simulink model "IEEE34bus_LeonardoEdit_Phasor_PI_ZIPload"  (R2024a)
settings: Solver=ode4  StartTime=0.0  StopTime=100  FixedStep=Ts  MaxStep=1e-4  RelTol=1e-4
InitFcn:
  | a=1; % Loading Factor
  | Ts=0.1;% For Delay Blocks in Voltage Regulator Controls
  | % phase to sequence conversion of RXB matrices
  | c=1*exp(sqrt(-1)*(120*pi/180));
  | T=[1 1 1;1 c*c c;1 c c*c];
  | Tinv=1/3*[1 1 1;1 c c*c;1 c*c c];
  | 
  | % Simulation data for the IEEE 34 Node Test Feeder model
  | mi2km = 1.60934;%  miles to km conversion
  | ft2km = 0.0003048; % feet to km conversion
  | ms2F = 1*1e-6/(2*pi*60);% microsiemens to Farads conversion
  | 
  | %% Configuration 300 - series reactance - ohm/mile
  | R_300 = [1.3368 0.2101 0.2130;0.2101 1.3238 0.2066;0.2130 0.2066 1.3294];
  | X_300 = [1.3343 0.5779 0.5015;0.5779 1.3569 0.4591;0.5015 0.4591 1.3471];
  | % charging susceptance - microsiemens/mile
  | B_300 = [5.3350 -1.5313 -0.9943;-1.5313 5.0979 -0.6212;-0.9943 -0.6212 4.8880];
  | 
  | R_300 = R_300/mi2km;
  | Rseq=Tinv*R_300*T;
  | R1_300=Rseq(2,2);R0_300=Rseq(1,1);
  | 
  | L_300 = (X_300/(2*pi*60))/mi2km;
  | Lseq=Tinv*L_300*T;
  | L1_300=Lseq(2,2);L0_300=Lseq(1,1);
  | 
  | C_300 =(B_300*ms2F)/mi2km;
  | Cseq=Tinv*C_300*T;
  | C1_300=Cseq(2,2);C0_300=Cseq(1,1);
  | 
  | %% Configuration 301 - series reactance - ohm/mile
  | R_301 = [1.9300 0.2327 0.2359;0.2327 1.9157 0.2288;0.2359 0.2288 1.9219];
  | X_301 = [1.4115 0.6442 0.5691;0.6442 1.4281 0.5238;0.5691 0.5238 1.4209];
  | % charging susceptance - microsiemens/mile
  | B_301 = [5.1207 -1.4364 -0.9402;-1.4364 4.9055 -0.5951;-0.9402 -0.5951 4.7154];
  | 
  | R_301 = R_301/mi2km;
  | Rseq=Tinv*R_301*T;
  | R1_301=Rseq(2,2);R0_301=Rseq(1,1);
  | 
  | L_301 = (X_301/(2*pi*60))/mi2km;
  | Lseq=Tinv*L_301*T;
  | L1_301=Lseq(2,2);L0_301=Lseq(1,1);
  | 
  | C_301 =(B_301*ms2F)/mi2km;
  | Cseq=Tinv*C_301*T;
  | C1_301=Cseq(2,2);C0_301=Cseq(1,1);
  | 
  | %% Configuration 302 - series reactance - ohm/mile
  | R_302 = [2.7995 0 0;0 0 0;0 0 0];
  | X_302 = [1.4855 0 0;0 0 0;0 0 0];
  | % charging susceptance - microsiemens/mile
  | B_302 = [4.2251 0 0;0 0 0;0 0 0];
  | 
  | R_302 = R_302/mi2km;
  | Rseq=Tinv*R_302*T;
  | R1_302=Rseq(2,2);R0_302=Rseq(1,1);
  | 
  | L_302 = (X_302/(2*pi*60))/mi2km;
  | Lseq=Tinv*L_302*T;
  | L1_302=Lseq(2,2);L0_302=Lseq(1,1);
  | 
  | C_302 =(B_302*ms2F)/mi2km;
  | Cseq=Tinv*C_302*T;
  | C1_302=Cseq(2,2);C0_302=Cseq(1,1);
  | 
  | %% Configuration 303 - series reactance - ohm/mile
  | R_303 = [0 0 0;0 2.7995 0;0 0 0];
  | X_303 = [0 0 0;0 1.4855 0;0 0 0];
  | % charging susceptance - microsiemens/mile
  | B_303 = [0 0 0;0 4.2251 0;0 0 0];
  | 
  | R_303 = R_303/mi2km;
  | Rseq=Tinv*R_303*T;
  | R1_303=Rseq(2,2);R0_303=Rseq(1,1);
  | 
  | L_303 = (X_303/(2*pi*60))/mi2km;
  | Lseq=Tinv*L_303*T;
  | L1_303=Lseq(2,2);L0_303=Lseq(1,1);
  | 
  | C_303 =(B_303*ms2F)/mi2km;
  | Cseq=Tinv*C_303*T;
  | C1_303=Cseq(2,2);C0_303=Cseq(1,1);
  | 
  | %% Configuration 303 - series reactance - ohm/mile
  | R_304 = [0 0 0;0 1.9217 0;0 0 0];
  | X_304 = [0 0 0;0 1.4212 0;0 0 0];
  | % charging susceptance - microsiemens/mile
  | B_304 = [0 0 0;0 4.3637 0;0 0 0];
  | 
  | R_304 = R_304/mi2km;
  | Rseq=Tinv*R_304*T;
  | R1_304=Rseq(2,2);R0_304=Rseq(1,1);
  | 
  | L_304 = (X_304/(2*pi*60))/mi2km;
  | Lseq=Tinv*L_304*T;
  | L1_304=Lseq(2,2);L0_304=Lseq(1,1);
  | 
  | C_304 =(B_304*ms2F)/mi2km;
  | Cseq=Tinv*C_304*T;
  | C1_304=Cseq(2,2);C0_304=Cseq(1,1);
undefined symbols (not defined in the file or in its folder): find_system, j
libraries: spsSeriesRLCBranchLib x157, spsGroundLib x103, spsVoltageMeasurementLib x100, spsControlledCurrentSourceLib x94, spsThreePhaseVIMeasurementLib x37, spsThreePhasePISectionLineLib x20, spsCurrentMeasurementLib x12, spsOnDelayLib x12, spsPiSectionLineLib x8, spsControlledVoltageSourceLib x6, spsDiscreteVariableTimeDelayLib x6, spsMutualInductanceLib x4
(part 1 of 8)
settings Model: ARTEMISmethode_block_infos=$$__separator__$$pi34variableloadwith3PV/ARTEMIS Guide$$__separator__$$  Creator=Arun  LastModifiedBy=leonardofdsantos
settings SolverCC: ShapePreserveControl=EnableAll  AlgebraicLoopSolver=TrustRegion  SolverResetMethod=Robust
settings DataIOCC: ReturnWorkspaceOutputs=off
settings DebuggingCC: ArithmeticOperatorsInVariantConditions=warning
settings ModelReferenceCC: EnableRefExpFcnMdlSchedulingChecks=on
settings SFSimCC: SimUseLocalCustomCode=off  CustomCodeUndefinedFunction=UseInterfaceOnly
settings RTWCC: RTWUseLocalCustomCode=off  GPUComputeCapability=3.5
settings CodeAppCC: StateflowObjectComments=on
settings SimscapeCC: SimscapeNormalizeSystem=off

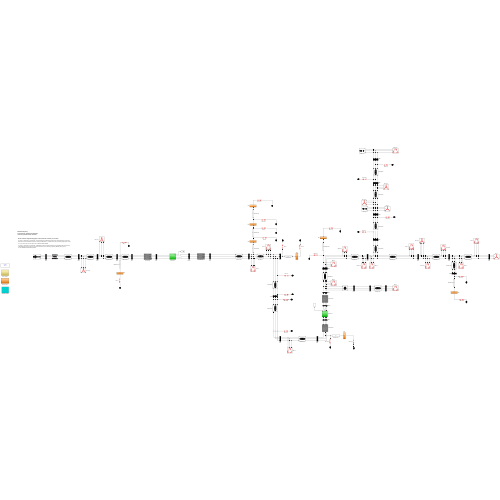
[thumbnail: Simulink's stored preview of the top-level diagram]
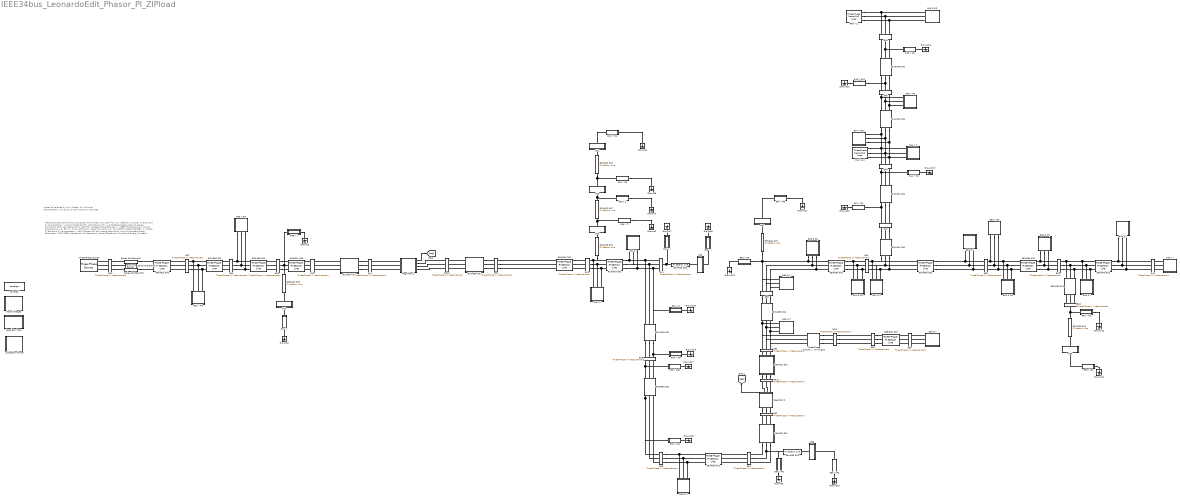
== system IEEE34bus_LeonardoEdit_Phasor_PI_ZIPload ==
  note: Model Developed by
      | Arun Suresh, Dr. Sukumar Kamalasadan,
      | University of North Carolina, Charlotte
  note: Please consider citing following papers if the model was useful for your research
      |
      | A. Suresh, R. Bisht and S. Kamalasadan, "A Coordinated Control Architecture With Inverter-Based Resources and Legacy
      | Controllers of Power Distribution System for Voltage Profile Balance," in IEEE Transactions on Industry Applications, vol. 58,
      | no. 5, pp. 6701-6712, Sept.-Oct. 2022, doi: 10.1109/TIA.2022.3183030.
      |
      | A. Suresh, R. Bisht and S. Kamalasadan, "ADMM Based LQR for Voltage Regulation Using Distributed Energy Resources,"
      | 2020 IEEE International Conference on Power Electronics, Drives and Energy Systems (PEDES), 2020, pp. 1-6,
      | doi: 10.1109/PEDES49360.2020.9379625.
  800 : spsThreePhaseVIMeasurementLib/Three-Phase V-I Measurement  VoltageMeasurement=phase-to-ground  SetLabelV=on  LabelV=V800  Vpu=off  VpuLL=off  CurrentMeasurement=yes  SetLabelI=on  LabelI=I800  Ipu=off  Pbase=100e6  Vbase=24900  OutputType=Complex  PhasorSimulation=on  PSBequivalent=0
  800-802 300 : spsThreePhasePISectionLineLib/Three-Phase PI Section Line  LConnTagsString=a|b|c  RConnTagsString=A|B|C  Length=2580*ft2km  Frequency=60  Resistances=[R1_300 R0_300]  Inductances=[L1_300 L0_300]  Capacitances=[C1_300 C0_300]
  802 : spsThreePhaseVIMeasurementLib/Three-Phase V-I Measurement  VoltageMeasurement=phase-to-ground  SetLabelV=on  LabelV=V802  Vpu=off  VpuLL=off  CurrentMeasurement=yes  SetLabelI=on  LabelI=I802  Ipu=off  Pbase=100e6  Vbase=24900  OutputType=Complex  PhasorSimulation=on  PSBequivalent=0
  802 Y PQ : Subsystem  mask(Three Phase Star ZIP Load (Phasor)){Vnom=24900, fnom=60, Pnom=[1e-6  30 25]*1e3/2 *a, Qnom=[0 15 14]*1e3/2 *a, LoadType=Constant P, Vlim=0.7}
      mask prompts: Vnom "Nominal Ph-Ph voltage (Vrms)"; fnom "Nominal Frequency fn (Hz)"; Pnom "Nominal Per Phase Active Power [Pa Pb Pc] (W)"; Qnom "Nominal Per Phase Reactive Power [Qa Qb Qc] (VAR)"; LoadType "Load Type"; Vlim "Minimum voltage (pu)"
      mask help:
      | Notes:
      | Three Phase Star Connected ZIP load model which gets converted to constant Z type if the voltage becomes lower than the Minimum Voltage.
      mask TypeOptions LoadType: Constant Z | Constant I | Constant P
      mask DialogControl ParameterTabVar0 Prompt: Parameters
      mask DialogControl ParameterTabVar01 Prompt: Type
      mask Display:
      | color('red');
      | %load figure 0deg
      | A=[-210,-180,-170,-160,-147,-140,-130,-120,-110,-80,-50,-49,-45,-39,-33,-26,-21,-18,-17,-19,-22,-22,-26,-27,-25,-22,-16,-9,-3,2,6,6,4,1,1,-3,-4,-2,2,7,14,20,26,29,30,28,24,24,21,20,21,25,31,37,44,49,50,50,80];
      | B=[-41.5,-41.5,-63,-20,-63,-20,-63,-20,-41.5,-41.5,-41.5,-34,-26,-21,-20,-22,-28,-37,-47,-57,-63,-63,-54,-44,-34,-26,-21,-20,-22,-28,-37,-47,-57,-63,-63,-54,-44,-34,-26,-21,-20,-22,-28,-37,-47,-57,-63,-63,-54,-44,-34,-26,-21,-20,-22,-28,-37,-41.50,-41.5];
      | % plot(A,B);
      | 
      | %load figure 0deg inverted
      | A1=[-80,-50,-49,-45,-39,-33,-26,-21,-18,-17,-19,-22,-22,-26,-27,-25,-22,-16,-9,-3,2,6,6,4,1,1,-3,-4,-2,2,7,14,20,26,29,30,28,24,24,21,20,21,25,31,37,44,49,50,50,80,110,120,130,143,150,160,170,180,210];
      | B1=[-41.5,-41.5,-34,-26,-21,-20,-22,-28,-37,-47,-57,-63,-63,-54,-44,-34,-26,-21,-20,-22,-28,-37,-47,-57,-63,-63,-54,-44,-34,-26,-21,-20,-22,-28,-37,-47,-57,-63,-63,-54,-44,-34,-26,-21,-20,-22,-28,-37,-41.5,-41.5,-41.5,-63,-20,-63,-20,-63,-20,-41.5,-41.5];
      | 
      | 
      | %load figure 90deg
      | C=[-41.5,-41.5,-20,-63,-20,-63,-20,-63,-41.5,-41.5,-41.5,-37,-28,-22,-20,-21,-26,-34,-44,-54,-63,-63,-57,-47,-37,-28,-22,-20,-21,-26,-34,-44,-54,-63,-63,-57,-47,-37,-28,-22,-20,-21,-26,-34,-44,-54,-63,-63,-57,-47,-37,-28,-22,-20,-21,-26,-34,-41.5,-41.5];
      | D=[190,160,150,140,130,123,110,100,90,80,50,50,49,44,37,31,25,21,20,21,24,24,28,30,29,26,20,14,7,2,-2,-4,-3,1,1,4,6,6,2,-3,-9,-16,-22,-25,-27,-26,-22,-22,-19,-17,-18,-21,-26,-33,-39,-45,-49,-50,-70];
      | plot(C,D);
      | 
      | 
      | %load figure -120deg
      | c=1*exp(sqrt(-1)*(-60*pi/180));
      | l=A1+j*B1;
      | m=l*c;
      | E=real(m);F=imag(m);
      | E=E+34.4400;F=F-118.53;
      | plot(E,F);
      | 
      | %load figure +120deg
      | c=1*exp(sqrt(-1)*(60*pi/180));
      | l=A+j*B;
      | m=l*c;
      | G=real(m);
      | H=imag(m);
      | G=G-117.44;H=H-118.5300;
      | plot(G,H);
      | 
      | color('black');
      | port_label('LConn', 1, 'A')
      | port_label('LConn', 2, 'B')
      | port_label('LConn', 3, 'C')
  802-806 300 : spsThreePhasePISectionLineLib/Three-Phase PI Section Line  LConnTagsString=a|b|c  RConnTagsString=A|B|C  Length=1730*ft2km  Frequency=60  Resistances=[R1_300 R0_300]  Inductances=[L1_300 L0_300]  Capacitances=[C1_300 C0_300]
  806 : spsThreePhaseVIMeasurementLib/Three-Phase V-I Measurement  VoltageMeasurement=phase-to-ground  SetLabelV=on  LabelV=V806  Vpu=off  VpuLL=off  CurrentMeasurement=yes  SetLabelI=on  LabelI=I806  Ipu=off  Pbase=100e6  Vbase=24900  OutputType=Complex  PhasorSimulation=on  PSBequivalent=0
  806 Y PQ : Subsystem  mask(Three Phase Star ZIP Load (Phasor)){Vnom=24900, fnom=60, Pnom=[1e-6  30 25]*1e3/2 *a, Qnom=[0 15 14]*1e3/2 *a, LoadType=Constant P, Vlim=0.7}
      mask prompts: Vnom "Nominal Ph-Ph voltage (Vrms)"; fnom "Nominal Frequency fn (Hz)"; Pnom "Nominal Per Phase Active Power [Pa Pb Pc] (W)"; Qnom "Nominal Per Phase Reactive Power [Qa Qb Qc] (VAR)"; LoadType "Load Type"; Vlim "Minimum voltage (pu)"
      mask help:
      | Notes:
      | Three Phase Star Connected ZIP load model which gets converted to constant Z type if the voltage becomes lower than the Minimum Voltage.
      mask TypeOptions LoadType: Constant Z | Constant I | Constant P
      mask DialogControl ParameterTabVar0 Prompt: Parameters
      mask DialogControl ParameterTabVar01 Prompt: Type
      mask Display:
      | color('red');
      | %load figure 0deg
      | A=[-210,-180,-170,-160,-147,-140,-130,-120,-110,-80,-50,-49,-45,-39,-33,-26,-21,-18,-17,-19,-22,-22,-26,-27,-25,-22,-16,-9,-3,2,6,6,4,1,1,-3,-4,-2,2,7,14,20,26,29,30,28,24,24,21,20,21,25,31,37,44,49,50,50,80];
      | B=[-41.5,-41.5,-63,-20,-63,-20,-63,-20,-41.5,-41.5,-41.5,-34,-26,-21,-20,-22,-28,-37,-47,-57,-63,-63,-54,-44,-34,-26,-21,-20,-22,-28,-37,-47,-57,-63,-63,-54,-44,-34,-26,-21,-20,-22,-28,-37,-47,-57,-63,-63,-54,-44,-34,-26,-21,-20,-22,-28,-37,-41.50,-41.5];
      | % plot(A,B);
      | 
      | %load figure 0deg inverted
      | A1=[-80,-50,-49,-45,-39,-33,-26,-21,-18,-17,-19,-22,-22,-26,-27,-25,-22,-16,-9,-3,2,6,6,4,1,1,-3,-4,-2,2,7,14,20,26,29,30,28,24,24,21,20,21,25,31,37,44,49,50,50,80,110,120,130,143,150,160,170,180,210];
      | B1=[-41.5,-41.5,-34,-26,-21,-20,-22,-28,-37,-47,-57,-63,-63,-54,-44,-34,-26,-21,-20,-22,-28,-37,-47,-57,-63,-63,-54,-44,-34,-26,-21,-20,-22,-28,-37,-47,-57,-63,-63,-54,-44,-34,-26,-21,-20,-22,-28,-37,-41.5,-41.5,-41.5,-63,-20,-63,-20,-63,-20,-41.5,-41.5];
      | 
      | 
      | %load figure 90deg
      | C=[-41.5,-41.5,-20,-63,-20,-63,-20,-63,-41.5,-41.5,-41.5,-37,-28,-22,-20,-21,-26,-34,-44,-54,-63,-63,-57,-47,-37,-28,-22,-20,-21,-26,-34,-44,-54,-63,-63,-57,-47,-37,-28,-22,-20,-21,-26,-34,-44,-54,-63,-63,-57,-47,-37,-28,-22,-20,-21,-26,-34,-41.5,-41.5];
      | D=[190,160,150,140,130,123,110,100,90,80,50,50,49,44,37,31,25,21,20,21,24,24,28,30,29,26,20,14,7,2,-2,-4,-3,1,1,4,6,6,2,-3,-9,-16,-22,-25,-27,-26,-22,-22,-19,-17,-18,-21,-26,-33,-39,-45,-49,-50,-70];
      | plot(C,D);
      | 
      | 
      | %load figure -120deg
      | c=1*exp(sqrt(-1)*(-60*pi/180));
      | l=A1+j*B1;
      | m=l*c;
      | E=real(m);F=imag(m);
      | E=E+34.4400;F=F-118.53;
      | plot(E,F);
      | 
      | %load figure +120deg
      | c=1*exp(sqrt(-1)*(60*pi/180));
      | l=A+j*B;
      | m=l*c;
      | G=real(m);
      | H=imag(m);
      | G=G-117.44;H=H-118.5300;
      | plot(G,H);
      | 
      | color('black');
      | port_label('LConn', 1, 'A')
      | port_label('LConn', 2, 'B')
      | port_label('LConn', 3, 'C')
  806-808 300 : spsThreePhasePISectionLineLib/Three-Phase PI Section Line  LConnTagsString=a|b|c  RConnTagsString=A|B|C  Length=32230*ft2km  Frequency=60  Resistances=[R1_300 R0_300]  Inductances=[L1_300 L0_300]  Capacitances=[C1_300 C0_300]
  808 : spsThreePhaseVIMeasurementLib/Three-Phase V-I Measurement  VoltageMeasurement=phase-to-ground  SetLabelV=on  LabelV=V808  Vpu=off  VpuLL=off  CurrentMeasurement=yes  SetLabelI=on  LabelI=I808  Ipu=off  Pbase=100e6  Vbase=24900  OutputType=Complex  PhasorSimulation=on  PSBequivalent=0
  808 Y I : Subsystem  mask(Single Phase ZIP Load){Vnom=1.0*14376.02, fnom=60, Pnom=16e3/2*a, Qnom=8e3/2*a, LoadType=constant I, Vlim=0.7}
      mask prompts: Vnom "Nominal Voltage Vn (Vrms)"; fnom "Nominal Frequency fn (Hz)"; Pnom "Nominal Active power (W)"; Qnom "Nominal Reactive power (VAR)"; LoadType "Load Type"; Vlim "Minimum voltage (pu)"
      mask help:
      | Notes:
      | Single Phase ZIP load model which gets converted to constant Z type if the voltage becomes lower than the Minimum Voltage.
      mask TypeOptions LoadType: Constant Z | constant I | constant P
      mask DialogControl ParameterTabVar0 Prompt: Parameters
      mask DialogControl ParameterTabVar1 Prompt: Type
      mask Display:
      | color('red');
      | A=[-210,-180,-170,-160,-147,-140,-130,-120,-110,-80,-50,-49,-45,-39,-33,-26,-21,-18,-17,-19,-22,-22,-26,-27,-25,-22,-16,-9,-3,2,6,6,4,1,1,-3,-4,-2,2,7,14,20,26,29,30,28,24,24,21,20,21,25,31,37,44,49,50,50,80];
      | B=[-41.5,-41.5,-63,-20,-63,-20,-63,-20,-41.5,-41.5,-41.5,-34,-26,-21,-20,-22,-28,-37,-47,-57,-63,-63,-54,-44,-34,-26,-21,-20,-22,-28,-37,-47,-57,-63,-63,-54,-44,-34,-26,-21,-20,-22,-28,-37,-47,-57,-63,-63,-54,-44,-34,-26,-21,-20,-22,-28,-37,-41.50,-41.5];
      | plot(A,B);
      | color('black');
      | port_label('LConn', 1, '+')
  808-810 303 : spsPiSectionLineLib/Pi Section Line  LConnTagsString=__new0  RConnTagsString=__new0  Phases=1  PiSections=1  Length=5804*ft2km  Frequency=60  Resistance=R1_303  Inductance=L1_303  Capacitance=C1_303  SpecifyConductance=off  Conductance=0  Measurements=None  Measurements2=None
      settings: LibrarySourceBlock=sps_lib/Power Grid Elements/Pi Section Line
  808-812 300 : spsThreePhasePISectionLineLib/Three-Phase PI Section Line  LConnTagsString=a|b|c  RConnTagsString=A|B|C  Length=37500*ft2km  Frequency=60  Resistances=[R1_300 R0_300]  Inductances=[L1_300 L0_300]  Capacitances=[C1_300 C0_300]
  810 : Subsystem
  810 Y I : Subsystem  mask(Single Phase ZIP Load){Vnom=1.0*14376.02, fnom=60, Pnom=16e3/2*a, Qnom=8e3/2*a, LoadType=constant I, Vlim=0.7}
      mask prompts: Vnom "Nominal Voltage Vn (Vrms)"; fnom "Nominal Frequency fn (Hz)"; Pnom "Nominal Active power (W)"; Qnom "Nominal Reactive power (VAR)"; LoadType "Load Type"; Vlim "Minimum voltage (pu)"
      mask help:
      | Notes:
      | Single Phase ZIP load model which gets converted to constant Z type if the voltage becomes lower than the Minimum Voltage.
      mask TypeOptions LoadType: Constant Z | constant I | constant P
      mask DialogControl ParameterTabVar0 Prompt: Parameters
      mask DialogControl ParameterTabVar1 Prompt: Type
      mask Display:
      | color('red');
      | A=[-210,-180,-170,-160,-147,-140,-130,-120,-110,-80,-50,-49,-45,-39,-33,-26,-21,-18,-17,-19,-22,-22,-26,-27,-25,-22,-16,-9,-3,2,6,6,4,1,1,-3,-4,-2,2,7,14,20,26,29,30,28,24,24,21,20,21,25,31,37,44,49,50,50,80];
      | B=[-41.5,-41.5,-63,-20,-63,-20,-63,-20,-41.5,-41.5,-41.5,-34,-26,-21,-20,-22,-28,-37,-47,-57,-63,-63,-54,-44,-34,-26,-21,-20,-22,-28,-37,-47,-57,-63,-63,-54,-44,-34,-26,-21,-20,-22,-28,-37,-47,-57,-63,-63,-54,-44,-34,-26,-21,-20,-22,-28,-37,-41.50,-41.5];
      | plot(A,B);
      | color('black');
      | port_label('LConn', 1, '+')
  812 : spsThreePhaseVIMeasurementLib/Three-Phase V-I Measurement  VoltageMeasurement=phase-to-ground  SetLabelV=on  LabelV=V812  Vpu=off  VpuLL=off  CurrentMeasurement=yes  SetLabelI=on  LabelI=I812  Ipu=off  Pbase=100e6  Vbase=24900  OutputType=Complex  PhasorSimulation=on  PSBequivalent=0
  812-814 300 : Subsystem  mask(Three-Phase PI Section Block){Rl=R_300, Ll=L_300, Cl=C_300, L=29730*ft2km}
      mask prompts: Rl "Resistance per unit Length(Ohm/Km)[3x3 matrix]"; Ll "Inductance per unit Length(H/Km)[3x3 matrix]"; Cl "Capacitance per unit Length(F/Km)[3x3 matrix]"; L "Length (Km)"
      mask help: This block models a three-phase transmission line with a single PI section.
  814 : spsThreePhaseVIMeasurementLib/Three-Phase V-I Measurement  VoltageMeasurement=phase-to-ground  SetLabelV=on  LabelV=V814  Vpu=off  VpuLL=off  CurrentMeasurement=yes  SetLabelI=on  LabelI=I814  Ipu=off  Pbase=100e6  Vbase=24900  OutputType=Complex  PhasorSimulation=on  PSBequivalent=0
  814-850 301 : Subsystem  mask(Three-Phase PI Section Block){Rl=R_301, Ll=L_301, Cl=C_301, L=10*ft2km}
      mask prompts: Rl "Resistance per unit Length(Ohm/Km)[3x3 matrix]"; Ll "Inductance per unit Length(H/Km)[3x3 matrix]"; Cl "Capacitance per unit Length(F/Km)[3x3 matrix]"; L "Length (Km)"
      mask help: This block models a three-phase transmission line with a single PI section.
  "816 " : spsThreePhaseVIMeasurementLib/Three-Phase V-I Measurement  VoltageMeasurement=phase-to-ground  SetLabelV=on  LabelV=V816  Vpu=off  VpuLL=off  CurrentMeasurement=yes  SetLabelI=on  LabelI=I816  Ipu=off  Pbase=100e6  Vbase=24900  OutputType=Complex  PhasorSimulation=on  PSBequivalent=0
  816 D I : Subsystem  mask(Three Phase Delta ZIP Load (Phasor)){Vnom=24900, fnom=60, Pnom=[1e-6  5 1e-6 ]*1e3/2 *a, Qnom=[0 2 0]*1e3/2 *a, LoadType=Constant I, Vlim=0.7}
      mask prompts: Vnom "Nominal Ph-Ph Voltage (Vrms)"; fnom "Nominal Frequency fn (Hz)"; Pnom "Nominal Per Phase Active Power [Pab Pbc Pca] (W)"; Qnom "Nominal Per Phase Reactive Power [Qab Qbc Qca] (VAR)"; LoadType "Load Type"; Vlim "Minimum Voltage (pu)"
      mask help:
      | Notes:
      | Three Phase Delta Connected ZIP load model which gets converted to constant Z type if the voltage becomes lower than the Minimum Voltage.
      mask TypeOptions LoadType: Constant Z | Constant I | Constant P
      mask DialogControl ParameterTabVar0 Prompt: Parameters
      mask DialogControl ParameterTabVar01 Prompt: Type
      mask Display:
      | color('red');
      | %load figure 0deg
      | A=[-210,-180,-170,-160,-147,-140,-130,-120,-110,-80,-50,-49,-45,-39,-33,-26,-21,-18,-17,-19,-22,-22,-26,-27,-25,-22,-16,-9,-3,2,6,6,4,1,1,-3,-4,-2,2,7,14,20,26,29,30,28,24,24,21,20,21,25,31,37,44,49,50,50,80];
      | B=[-41.5,-41.5,-63,-20,-63,-20,-63,-20,-41.5,-41.5,-41.5,-34,-26,-21,-20,-22,-28,-37,-47,-57,-63,-63,-54,-44,-34,-26,-21,-20,-22,-28,-37,-47,-57,-63,-63,-54,-44,-34,-26,-21,-20,-22,-28,-37,-47,-57,-63,-63,-54,-44,-34,-26,-21,-20,-22,-28,-37,-41.50,-41.5];
      | plot(A,B);
      | 
      | %load figure 0deg inverted
      | A1=[-80,-50,-49,-45,-39,-33,-26,-21,-18,-17,-19,-22,-22,-26,-27,-25,-22,-16,-9,-3,2,6,6,4,1,1,-3,-4,-2,2,7,14,20,26,29,30,28,24,24,21,20,21,25,31,37,44,49,50,50,80,110,120,130,143,150,160,170,180,210];
      | B1=[-41.5,-41.5,-34,-26,-21,-20,-22,-28,-37,-47,-57,-63,-63,-54,-44,-34,-26,-21,-20,-22,-28,-37,-47,-57,-63,-63,-54,-44,-34,-26,-21,-20,-22,-28,-37,-47,-57,-63,-63,-54,-44,-34,-26,-21,-20,-22,-28,-37,-41.5,-41.5,-41.5,-63,-20,-63,-20,-63,-20,-41.5,-41.5];
      | 
      | 
      | %load figure -120deg
      | c=1*exp(sqrt(-1)*(-60*pi/180));
      | l=A1+j*B1;
      | m=l*c;
      | E=real(m);F=imag(m);
      | E=E+10.94;F=F+161.1;
      | plot(E,F);
      | 
      | %load figure +120deg
      | c=1*exp(sqrt(-1)*(60*pi/180));
      | l=A1+j*B1;
      | m=l*c;
      | G=real(m);
      | H=imag(m);
      | G=G-205.94;H=H+48.53;
      | plot(G,H);
      | 
      | color('black');
      | port_label('LConn', 1, 'A')
      | port_label('LConn', 2, 'B')
      | port_label('LConn', 3, 'C')
  816-818 302 : spsPiSectionLineLib/Pi Section Line  LConnTagsString=__new0  RConnTagsString=__new0  Phases=1  PiSections=1  Length=1710*ft2km  Frequency=60  Resistance=R1_302  Inductance=L1_302  Capacitance=C1_302  SpecifyConductance=off  Conductance=0  Measurements=None  Measurements2=None
      settings: LibrarySourceBlock=sps_lib/Power Grid Elements/Pi Section Line
  816-824 301 : spsThreePhasePISectionLineLib/Three-Phase PI Section Line  LConnTagsString=a|b|c  RConnTagsString=A|B|C  Length=10210*ft2km  Frequency=60  Resistances=[R1_301 R0_301]  Inductances=[L1_301 L0_301]  Capacitances=[C1_301 C0_301]
  818 : Subsystem
  818 Y Z : Subsystem  mask(Single Phase ZIP Load){Vnom=1.0*14376.02, fnom=60, Pnom=34e3/2 *a, Qnom=17e3/2*a, LoadType=Constant Z, Vlim=0.7}
      mask prompts: Vnom "Nominal Voltage Vn (Vrms)"; fnom "Nominal Frequency fn (Hz)"; Pnom "Nominal Active power (W)"; Qnom "Nominal Reactive power (VAR)"; LoadType "Load Type"; Vlim "Minimum voltage (pu)"
      mask help:
      | Notes:
      | Single Phase ZIP load model which gets converted to constant Z type if the voltage becomes lower than the Minimum Voltage.
      mask TypeOptions LoadType: Constant Z | constant I | constant P
      mask DialogControl ParameterTabVar0 Prompt: Parameters
      mask DialogControl ParameterTabVar1 Prompt: Type
      mask Display:
      | color('red');
      | A=[-210,-180,-170,-160,-147,-140,-130,-120,-110,-80,-50,-49,-45,-39,-33,-26,-21,-18,-17,-19,-22,-22,-26,-27,-25,-22,-16,-9,-3,2,6,6,4,1,1,-3,-4,-2,2,7,14,20,26,29,30,28,24,24,21,20,21,25,31,37,44,49,50,50,80];
      | B=[-41.5,-41.5,-63,-20,-63,-20,-63,-20,-41.5,-41.5,-41.5,-34,-26,-21,-20,-22,-28,-37,-47,-57,-63,-63,-54,-44,-34,-26,-21,-20,-22,-28,-37,-47,-57,-63,-63,-54,-44,-34,-26,-21,-20,-22,-28,-37,-47,-57,-63,-63,-54,-44,-34,-26,-21,-20,-22,-28,-37,-41.50,-41.5];
      | plot(A,B);
      | color('black');
      | port_label('LConn', 1, '+')
  818-820 302 : spsPiSectionLineLib/Pi Section Line  LConnTagsString=__new0  RConnTagsString=__new0  Phases=1  PiSections=1  Length=48150*ft2km  Frequency=60  Resistance=R1_302  Inductance=L1_302  Capacitance=C1_302  SpecifyConductance=off  Conductance=0  Measurements=None  Measurements2=None
      settings: LibrarySourceBlock=sps_lib/Power Grid Elements/Pi Section Line
  820 : Subsystem
  820 Y PQ : Subsystem  mask(Single Phase ZIP Load){Vnom=1.0*14376.02, fnom=60, Pnom=135e3/2 *a, Qnom=70e3/2*a, LoadType=constant P, Vlim=0.7}
      mask prompts: Vnom "Nominal Voltage Vn (Vrms)"; fnom "Nominal Frequency fn (Hz)"; Pnom "Nominal Active power (W)"; Qnom "Nominal Reactive power (VAR)"; LoadType "Load Type"; Vlim "Minimum voltage (pu)"
      mask help:
      | Notes:
      | Single Phase ZIP load model which gets converted to constant Z type if the voltage becomes lower than the Minimum Voltage.
      mask TypeOptions LoadType: Constant Z | constant I | constant P
      mask DialogControl ParameterTabVar0 Prompt: Parameters
      mask DialogControl ParameterTabVar1 Prompt: Type
      mask Display:
      | color('red');
      | A=[-210,-180,-170,-160,-147,-140,-130,-120,-110,-80,-50,-49,-45,-39,-33,-26,-21,-18,-17,-19,-22,-22,-26,-27,-25,-22,-16,-9,-3,2,6,6,4,1,1,-3,-4,-2,2,7,14,20,26,29,30,28,24,24,21,20,21,25,31,37,44,49,50,50,80];
      | B=[-41.5,-41.5,-63,-20,-63,-20,-63,-20,-41.5,-41.5,-41.5,-34,-26,-21,-20,-22,-28,-37,-47,-57,-63,-63,-54,-44,-34,-26,-21,-20,-22,-28,-37,-47,-57,-63,-63,-54,-44,-34,-26,-21,-20,-22,-28,-37,-47,-57,-63,-63,-54,-44,-34,-26,-21,-20,-22,-28,-37,-41.50,-41.5];
      | plot(A,B);
      | color('black');
      | port_label('LConn', 1, '+')
  820-822 302 : spsPiSectionLineLib/Pi Section Line  LConnTagsString=__new0  RConnTagsString=__new0  Phases=1  PiSections=1  Length=13740*ft2km  Frequency=60  Resistance=R1_302  Inductance=L1_302  Capacitance=C1_302  SpecifyConductance=off  Conductance=0  Measurements=None  Measurements2=None
      settings: LibrarySourceBlock=sps_lib/Power Grid Elements/Pi Section Line
  820Y Z : Subsystem  mask(Single Phase ZIP Load){Vnom=1.0*14376.02, fnom=60, Pnom=34e3/2 *a, Qnom=17e3/2*a, LoadType=Constant Z, Vlim=0.7}
      mask prompts: Vnom "Nominal Voltage Vn (Vrms)"; fnom "Nominal Frequency fn (Hz)"; Pnom "Nominal Active power (W)"; Qnom "Nominal Reactive power (VAR)"; LoadType "Load Type"; Vlim "Minimum voltage (pu)"
      mask help:
      | Notes:
      | Single Phase ZIP load model which gets converted to constant Z type if the voltage becomes lower than the Minimum Voltage.
      mask TypeOptions LoadType: Constant Z | constant I | constant P
      mask DialogControl ParameterTabVar0 Prompt: Parameters
      mask DialogControl ParameterTabVar1 Prompt: Type
      mask Display:
      | color('red');
      | A=[-210,-180,-170,-160,-147,-140,-130,-120,-110,-80,-50,-49,-45,-39,-33,-26,-21,-18,-17,-19,-22,-22,-26,-27,-25,-22,-16,-9,-3,2,6,6,4,1,1,-3,-4,-2,2,7,14,20,26,29,30,28,24,24,21,20,21,25,31,37,44,49,50,50,80];
      | B=[-41.5,-41.5,-63,-20,-63,-20,-63,-20,-41.5,-41.5,-41.5,-34,-26,-21,-20,-22,-28,-37,-47,-57,-63,-63,-54,-44,-34,-26,-21,-20,-22,-28,-37,-47,-57,-63,-63,-54,-44,-34,-26,-21,-20,-22,-28,-37,-47,-57,-63,-63,-54,-44,-34,-26,-21,-20,-22,-28,-37,-41.50,-41.5];
      | plot(A,B);
      | color('black');
      | port_label('LConn', 1, '+')
  822 : Subsystem
  822 Y PQ : Subsystem  mask(Single Phase ZIP Load){Vnom=1.0*14376.02, fnom=60, Pnom=135e3/2 *a, Qnom=70e3/2*a, LoadType=constant P, Vlim=0.7}
      mask prompts: Vnom "Nominal Voltage Vn (Vrms)"; fnom "Nominal Frequency fn (Hz)"; Pnom "Nominal Active power (W)"; Qnom "Nominal Reactive power (VAR)"; LoadType "Load Type"; Vlim "Minimum voltage (pu)"
      mask help:
      | Notes:
      | Single Phase ZIP load model which gets converted to constant Z type if the voltage becomes lower than the Minimum Voltage.
      mask TypeOptions LoadType: Constant Z | constant I | constant P
      mask DialogControl ParameterTabVar0 Prompt: Parameters
      mask DialogControl ParameterTabVar1 Prompt: Type
      mask Display:
      | color('red');
      | A=[-210,-180,-170,-160,-147,-140,-130,-120,-110,-80,-50,-49,-45,-39,-33,-26,-21,-18,-17,-19,-22,-22,-26,-27,-25,-22,-16,-9,-3,2,6,6,4,1,1,-3,-4,-2,2,7,14,20,26,29,30,28,24,24,21,20,21,25,31,37,44,49,50,50,80];
      | B=[-41.5,-41.5,-63,-20,-63,-20,-63,-20,-41.5,-41.5,-41.5,-34,-26,-21,-20,-22,-28,-37,-47,-57,-63,-63,-54,-44,-34,-26,-21,-20,-22,-28,-37,-47,-57,-63,-63,-54,-44,-34,-26,-21,-20,-22,-28,-37,-47,-57,-63,-63,-54,-44,-34,-26,-21,-20,-22,-28,-37,-41.50,-41.5];
      | plot(A,B);
      | color('black');
      | port_label('LConn', 1, '+')
  "824 " : spsThreePhaseVIMeasurementLib/Three-Phase V-I Measurement  VoltageMeasurement=phase-to-ground  SetLabelV=on  LabelV=V824  Vpu=off  VpuLL=off  CurrentMeasurement=yes  SetLabelI=on  LabelI=I824  Ipu=off  Pbase=100e6  Vbase=24900  OutputType=Complex  PhasorSimulation=on  PSBequivalent=0
  824 D I : Subsystem  mask(Three Phase Delta ZIP Load (Phasor)){Vnom=24900, fnom=60, Pnom=[1e-3  5 1e-3 ]*1e3/2 *a, Qnom=[0 2 0]*1e3/2 *a, LoadType=Constant I, Vlim=0.7}
      mask prompts: Vnom "Nominal Ph-Ph Voltage (Vrms)"; fnom "Nominal Frequency fn (Hz)"; Pnom "Nominal Per Phase Active Power [Pab Pbc Pca] (W)"; Qnom "Nominal Per Phase Reactive Power [Qab Qbc Qca] (VAR)"; LoadType "Load Type"; Vlim "Minimum Voltage (pu)"
      mask help:
      | Notes:
      | Three Phase Delta Connected ZIP load model which gets converted to constant Z type if the voltage becomes lower than the Minimum Voltage.
      mask TypeOptions LoadType: Constant Z | Constant I | Constant P
      mask DialogControl ParameterTabVar0 Prompt: Parameters
      mask DialogControl ParameterTabVar01 Prompt: Type
      mask Display:
      | color('red');
      | %load figure 0deg
      | A=[-210,-180,-170,-160,-147,-140,-130,-120,-110,-80,-50,-49,-45,-39,-33,-26,-21,-18,-17,-19,-22,-22,-26,-27,-25,-22,-16,-9,-3,2,6,6,4,1,1,-3,-4,-2,2,7,14,20,26,29,30,28,24,24,21,20,21,25,31,37,44,49,50,50,80];
      | B=[-41.5,-41.5,-63,-20,-63,-20,-63,-20,-41.5,-41.5,-41.5,-34,-26,-21,-20,-22,-28,-37,-47,-57,-63,-63,-54,-44,-34,-26,-21,-20,-22,-28,-37,-47,-57,-63,-63,-54,-44,-34,-26,-21,-20,-22,-28,-37,-47,-57,-63,-63,-54,-44,-34,-26,-21,-20,-22,-28,-37,-41.50,-41.5];
      | plot(A,B);
      | 
      | %load figure 0deg inverted
      | A1=[-80,-50,-49,-45,-39,-33,-26,-21,-18,-17,-19,-22,-22,-26,-27,-25,-22,-16,-9,-3,2,6,6,4,1,1,-3,-4,-2,2,7,14,20,26,29,30,28,24,24,21,20,21,25,31,37,44,49,50,50,80,110,120,130,143,150,160,170,180,210];
      | B1=[-41.5,-41.5,-34,-26,-21,-20,-22,-28,-37,-47,-57,-63,-63,-54,-44,-34,-26,-21,-20,-22,-28,-37,-47,-57,-63,-63,-54,-44,-34,-26,-21,-20,-22,-28,-37,-47,-57,-63,-63,-54,-44,-34,-26,-21,-20,-22,-28,-37,-41.5,-41.5,-41.5,-63,-20,-63,-20,-63,-20,-41.5,-41.5];
      | 
      | 
      | %load figure -120deg
      | c=1*exp(sqrt(-1)*(-60*pi/180));
      | l=A1+j*B1;
      | m=l*c;
      | E=real(m);F=imag(m);
      | E=E+10.94;F=F+161.1;
      | plot(E,F);
      | 
      | %load figure +120deg
      | c=1*exp(sqrt(-1)*(60*pi/180));
      | l=A1+j*B1;
      | m=l*c;
      | G=real(m);
      | H=imag(m);
      | G=G-205.94;H=H+48.53;
      | plot(G,H);
      | 
      | color('black');
      | port_label('LConn', 1, 'A')
      | port_label('LConn', 2, 'B')
      | port_label('LConn', 3, 'C')
  824 Y I : Subsystem  mask(Single Phase ZIP Load){Vnom=1.0*14376.02, fnom=60, Pnom=40e3/2 *a, Qnom=20e3/2*a, LoadType=constant I, Vlim=0.7}
      mask prompts: Vnom "Nominal Voltage Vn (Vrms)"; fnom "Nominal Frequency fn (Hz)"; Pnom "Nominal Active power (W)"; Qnom "Nominal Reactive power (VAR)"; LoadType "Load Type"; Vlim "Minimum voltage (pu)"
      mask help:
      | Notes:
      | Single Phase ZIP load model which gets converted to constant Z type if the voltage becomes lower than the Minimum Voltage.
      mask TypeOptions LoadType: Constant Z | constant I | constant P
      mask DialogControl ParameterTabVar0 Prompt: Parameters
      mask DialogControl ParameterTabVar1 Prompt: Type
      mask Display:
      | color('red');
      | A=[-210,-180,-170,-160,-147,-140,-130,-120,-110,-80,-50,-49,-45,-39,-33,-26,-21,-18,-17,-19,-22,-22,-26,-27,-25,-22,-16,-9,-3,2,6,6,4,1,1,-3,-4,-2,2,7,14,20,26,29,30,28,24,24,21,20,21,25,31,37,44,49,50,50,80];
      | B=[-41.5,-41.5,-63,-20,-63,-20,-63,-20,-41.5,-41.5,-41.5,-34,-26,-21,-20,-22,-28,-37,-47,-57,-63,-63,-54,-44,-34,-26,-21,-20,-22,-28,-37,-47,-57,-63,-63,-54,-44,-34,-26,-21,-20,-22,-28,-37,-47,-57,-63,-63,-54,-44,-34,-26,-21,-20,-22,-28,-37,-41.50,-41.5];
      | plot(A,B);
      | color('black');
      | port_label('LConn', 1, '+')
  824-826 303 : spsPiSectionLineLib/Pi Section Line  LConnTagsString=__new0  RConnTagsString=__new0  Phases=1  PiSections=1  Length=3030*ft2km  Frequency=60  Resistance=R1_303  Inductance=L1_303  Capacitance=C1_303  SpecifyConductance=off  Conductance=0  Measurements=None  Measurements2=None
      settings: LibrarySourceBlock=sps_lib/Power Grid Elements/Pi Section Line
  824-828 301 : spsThreePhasePISectionLineLib/Three-Phase PI Section Line  LConnTagsString=a|b|c  RConnTagsString=A|B|C  Length=840*ft2km  Frequency=60  Resistances=[R1_301 R0_301]  Inductances=[L1_301 L0_301]  Capacitances=[C1_301 C0_301]
  826 : Subsystem
  826 Y I : Subsystem  mask(Single Phase ZIP Load){Vnom=1.0*14376.02, fnom=60, Pnom=40e3/2 *a, Qnom=20e3/2*a, LoadType=constant I, Vlim=0.7}
      mask prompts: Vnom "Nominal Voltage Vn (Vrms)"; fnom "Nominal Frequency fn (Hz)"; Pnom "Nominal Active power (W)"; Qnom "Nominal Reactive power (VAR)"; LoadType "Load Type"; Vlim "Minimum voltage (pu)"
      mask help:
      | Notes:
      | Single Phase ZIP load model which gets converted to constant Z type if the voltage becomes lower than the Minimum Voltage.
      mask TypeOptions LoadType: Constant Z | constant I | constant P
      mask DialogControl ParameterTabVar0 Prompt: Parameters
      mask DialogControl ParameterTabVar1 Prompt: Type
      mask Display:
      | color('red');
      | A=[-210,-180,-170,-160,-147,-140,-130,-120,-110,-80,-50,-49,-45,-39,-33,-26,-21,-18,-17,-19,-22,-22,-26,-27,-25,-22,-16,-9,-3,2,6,6,4,1,1,-3,-4,-2,2,7,14,20,26,29,30,28,24,24,21,20,21,25,31,37,44,49,50,50,80];
      | B=[-41.5,-41.5,-63,-20,-63,-20,-63,-20,-41.5,-41.5,-41.5,-34,-26,-21,-20,-22,-28,-37,-47,-57,-63,-63,-54,-44,-34,-26,-21,-20,-22,-28,-37,-47,-57,-63,-63,-54,-44,-34,-26,-21,-20,-22,-28,-37,-47,-57,-63,-63,-54,-44,-34,-26,-21,-20,-22,-28,-37,-41.50,-41.5];
      | plot(A,B);
      | color('black');
      | port_label('LConn', 1, '+')
  826 Y I1 : Subsystem  mask(Single Phase ZIP Load){Vnom=1.0*14376.02, fnom=60, Pnom=40e3/2 *a, Qnom=20e3/2*a, LoadType=constant I, Vlim=0.7}
      mask prompts: Vnom "Nominal Voltage Vn (Vrms)"; fnom "Nominal Frequency fn (Hz)"; Pnom "Nominal Active power (W)"; Qnom "Nominal Reactive power (VAR)"; LoadType "Load Type"; Vlim "Minimum voltage (pu)"
      mask help:
      | Notes:
      | Single Phase ZIP load model which gets converted to constant Z type if the voltage becomes lower than the Minimum Voltage.
      mask TypeOptions LoadType: Constant Z | constant I | constant P
      mask DialogControl ParameterTabVar0 Prompt: Parameters
      mask DialogControl ParameterTabVar1 Prompt: Type
      mask Display:
      | color('red');
      | A=[-210,-180,-170,-160,-147,-140,-130,-120,-110,-80,-50,-49,-45,-39,-33,-26,-21,-18,-17,-19,-22,-22,-26,-27,-25,-22,-16,-9,-3,2,6,6,4,1,1,-3,-4,-2,2,7,14,20,26,29,30,28,24,24,21,20,21,25,31,37,44,49,50,50,80];
      | B=[-41.5,-41.5,-63,-20,-63,-20,-63,-20,-41.5,-41.5,-41.5,-34,-26,-21,-20,-22,-28,-37,-47,-57,-63,-63,-54,-44,-34,-26,-21,-20,-22,-28,-37,-47,-57,-63,-63,-54,-44,-34,-26,-21,-20,-22,-28,-37,-47,-57,-63,-63,-54,-44,-34,-26,-21,-20,-22,-28,-37,-41.50,-41.5];
      | plot(A,B);
      | color('black');
      | port_label('LConn', 1, '+')
  828 : spsThreePhaseVIMeasurementLib/Three-Phase V-I Measurement  VoltageMeasurement=phase-to-ground  SetLabelV=on  LabelV=V828  Vpu=off  VpuLL=off  CurrentMeasurement=yes  SetLabelI=on  LabelI=I828  Ipu=off  Pbase=100e6  Vbase=24900  OutputType=Complex  PhasorSimulation=on  PSBequivalent=0
  828 Y PQ : Subsystem  mask(Single Phase ZIP Load){Vnom=1.0*14376.02, fnom=60, Pnom=4e3/2 *a, Qnom=2e3/2 *a, LoadType=constant P, Vlim=0.7}
      mask prompts: Vnom "Nominal Voltage Vn (Vrms)"; fnom "Nominal Frequency fn (Hz)"; Pnom "Nominal Active power (W)"; Qnom "Nominal Reactive power (VAR)"; LoadType "Load Type"; Vlim "Minimum voltage (pu)"
      mask help:
      | Notes:
      | Single Phase ZIP load model which gets converted to constant Z type if the voltage becomes lower than the Minimum Voltage.
      mask TypeOptions LoadType: Constant Z | constant I | constant P
      mask DialogControl ParameterTabVar0 Prompt: Parameters
      mask DialogControl ParameterTabVar1 Prompt: Type
      mask Display:
      | color('red');
      | A=[-210,-180,-170,-160,-147,-140,-130,-120,-110,-80,-50,-49,-45,-39,-33,-26,-21,-18,-17,-19,-22,-22,-26,-27,-25,-22,-16,-9,-3,2,6,6,4,1,1,-3,-4,-2,2,7,14,20,26,29,30,28,24,24,21,20,21,25,31,37,44,49,50,50,80];
      | B=[-41.5,-41.5,-63,-20,-63,-20,-63,-20,-41.5,-41.5,-41.5,-34,-26,-21,-20,-22,-28,-37,-47,-57,-63,-63,-54,-44,-34,-26,-21,-20,-22,-28,-37,-47,-57,-63,-63,-54,-44,-34,-26,-21,-20,-22,-28,-37,-47,-57,-63,-63,-54,-44,-34,-26,-21,-20,-22,-28,-37,-41.50,-41.5];
      | plot(A,B);
      | color('black');
      | port_label('LConn', 1, '+')
  828 Y PQ1 : Subsystem  mask(Single Phase ZIP Load){Vnom=1.0*14376.02, fnom=60, Pnom=7*1e3/2 *a, Qnom=3*1e3/2 *a, LoadType=constant P, Vlim=0.7}
      mask prompts: Vnom "Nominal Voltage Vn (Vrms)"; fnom "Nominal Frequency fn (Hz)"; Pnom "Nominal Active power (W)"; Qnom "Nominal Reactive power (VAR)"; LoadType "Load Type"; Vlim "Minimum voltage (pu)"
      mask help:
      | Notes:
      | Single Phase ZIP load model which gets converted to constant Z type if the voltage becomes lower than the Minimum Voltage.
      mask TypeOptions LoadType: Constant Z | constant I | constant P
      mask DialogControl ParameterTabVar0 Prompt: Parameters
      mask DialogControl ParameterTabVar1 Prompt: Type
      mask Display:
      | color('red');
      | A=[-210,-180,-170,-160,-147,-140,-130,-120,-110,-80,-50,-49,-45,-39,-33,-26,-21,-18,-17,-19,-22,-22,-26,-27,-25,-22,-16,-9,-3,2,6,6,4,1,1,-3,-4,-2,2,7,14,20,26,29,30,28,24,24,21,20,21,25,31,37,44,49,50,50,80];
      | B=[-41.5,-41.5,-63,-20,-63,-20,-63,-20,-41.5,-41.5,-41.5,-34,-26,-21,-20,-22,-28,-37,-47,-57,-63,-63,-54,-44,-34,-26,-21,-20,-22,-28,-37,-47,-57,-63,-63,-54,-44,-34,-26,-21,-20,-22,-28,-37,-47,-57,-63,-63,-54,-44,-34,-26,-21,-20,-22,-28,-37,-41.50,-41.5];
      | plot(A,B);
      | color('black');
      | port_label('LConn', 1, '+')
  828-830 301 : spsThreePhasePISectionLineLib/Three-Phase PI Section Line  LConnTagsString=a|b|c  RConnTagsString=A|B|C  Length=20440*ft2km  Frequency=60  Resistances=[R1_301 R0_301]  Inductances=[L1_301 L0_301]  Capacitances=[C1_301 C0_301]
  830 : spsThreePhaseVIMeasurementLib/Three-Phase V-I Measurement  VoltageMeasurement=phase-to-ground  SetLabelV=on  LabelV=V830  Vpu=off  VpuLL=off  CurrentMeasurement=no  SetLabelI=on  LabelI=I830  Ipu=off  Pbase=100e6  Vbase=24900  OutputType=Complex  PhasorSimulation=on  PSBequivalent=0
  830 D Z : Subsystem  mask(Three Phase Delta ZIP Load (Phasor)){Vnom=24900, fnom=60, Pnom=[10 10 25]*1e3 *a, Qnom=[5 5 10]*1e3 *a, LoadType=Constant Z, Vlim=0.7}
      mask prompts: Vnom "Nominal Ph-Ph Voltage (Vrms)"; fnom "Nominal Frequency fn (Hz)"; Pnom "Nominal Per Phase Active Power [Pab Pbc Pca] (W)"; Qnom "Nominal Per Phase Reactive Power [Qab Qbc Qca] (VAR)"; LoadType "Load Type"; Vlim "Minimum Voltage (pu)"
      mask help:
      | Notes:
      | Three Phase Delta Connected ZIP load model which gets converted to constant Z type if the voltage becomes lower than the Minimum Voltage.
      mask TypeOptions LoadType: Constant Z | Constant I | Constant P
      mask DialogControl ParameterTabVar0 Prompt: Parameters
      mask DialogControl ParameterTabVar01 Prompt: Type
      mask Display:
      | color('red');
      | %load figure 0deg
      | A=[-210,-180,-170,-160,-147,-140,-130,-120,-110,-80,-50,-49,-45,-39,-33,-26,-21,-18,-17,-19,-22,-22,-26,-27,-25,-22,-16,-9,-3,2,6,6,4,1,1,-3,-4,-2,2,7,14,20,26,29,30,28,24,24,21,20,21,25,31,37,44,49,50,50,80];
      | B=[-41.5,-41.5,-63,-20,-63,-20,-63,-20,-41.5,-41.5,-41.5,-34,-26,-21,-20,-22,-28,-37,-47,-57,-63,-63,-54,-44,-34,-26,-21,-20,-22,-28,-37,-47,-57,-63,-63,-54,-44,-34,-26,-21,-20,-22,-28,-37,-47,-57,-63,-63,-54,-44,-34,-26,-21,-20,-22,-28,-37,-41.50,-41.5];
      | plot(A,B);
      | 
      | %load figure 0deg inverted
      | A1=[-80,-50,-49,-45,-39,-33,-26,-21,-18,-17,-19,-22,-22,-26,-27,-25,-22,-16,-9,-3,2,6,6,4,1,1,-3,-4,-2,2,7,14,20,26,29,30,28,24,24,21,20,21,25,31,37,44,49,50,50,80,110,120,130,143,150,160,170,180,210];
      | B1=[-41.5,-41.5,-34,-26,-21,-20,-22,-28,-37,-47,-57,-63,-63,-54,-44,-34,-26,-21,-20,-22,-28,-37,-47,-57,-63,-63,-54,-44,-34,-26,-21,-20,-22,-28,-37,-47,-57,-63,-63,-54,-44,-34,-26,-21,-20,-22,-28,-37,-41.5,-41.5,-41.5,-63,-20,-63,-20,-63,-20,-41.5,-41.5];
      | 
      | 
      | %load figure -120deg
      | c=1*exp(sqrt(-1)*(-60*pi/180));
      | l=A1+j*B1;
      | m=l*c;
      | E=real(m);F=imag(m);
      | E=E+10.94;F=F+161.1;
      | plot(E,F);
      | 
      | %load figure +120deg
      | c=1*exp(sqrt(-1)*(60*pi/180));
      | l=A1+j*B1;
      | m=l*c;
      | G=real(m);
      | H=imag(m);
      | G=G-205.94;H=H+48.53;
      | plot(G,H);
      | 
      | color('black');
      | port_label('LConn', 1, 'A')
      | port_label('LConn', 2, 'B')
      | port_label('LConn', 3, 'C')
  830 Y PQ : Subsystem  mask(Single Phase ZIP Load){Vnom=1.0*14376.02, fnom=60, Pnom=7e3/2 *a, Qnom=3e3/2 *a, LoadType=constant P, Vlim=0.7}
      mask prompts: Vnom "Nominal Voltage Vn (Vrms)"; fnom "Nominal Frequency fn (Hz)"; Pnom "Nominal Active power (W)"; Qnom "Nominal Reactive power (VAR)"; LoadType "Load Type"; Vlim "Minimum voltage (pu)"
      mask help:
      | Notes:
      | Single Phase ZIP load model which gets converted to constant Z type if the voltage becomes lower than the Minimum Voltage.
      mask TypeOptions LoadType: Constant Z | constant I | constant P
      mask DialogControl ParameterTabVar0 Prompt: Parameters
      mask DialogControl ParameterTabVar1 Prompt: Type
      mask Display:
      | color('red');
      | A=[-210,-180,-170,-160,-147,-140,-130,-120,-110,-80,-50,-49,-45,-39,-33,-26,-21,-18,-17,-19,-22,-22,-26,-27,-25,-22,-16,-9,-3,2,6,6,4,1,1,-3,-4,-2,2,7,14,20,26,29,30,28,24,24,21,20,21,25,31,37,44,49,50,50,80];
      | B=[-41.5,-41.5,-63,-20,-63,-20,-63,-20,-41.5,-41.5,-41.5,-34,-26,-21,-20,-22,-28,-37,-47,-57,-63,-63,-54,-44,-34,-26,-21,-20,-22,-28,-37,-47,-57,-63,-63,-54,-44,-34,-26,-21,-20,-22,-28,-37,-47,-57,-63,-63,-54,-44,-34,-26,-21,-20,-22,-28,-37,-41.50,-41.5];
      | plot(A,B);
      | color('black');
      | port_label('LConn', 1, '+')
  830-854 301 : spsThreePhasePISectionLineLib/Three-Phase PI Section Line  LConnTagsString=a|b|c  RConnTagsString=A|B|C  Length=520*ft2km  Frequency=60  Resistances=[R1_301 R0_301]  Inductances=[L1_301 L0_301]  Capacitances=[C1_301 C0_301]
  832 : spsThreePhaseVIMeasurementLib/Three-Phase V-I Measurement  VoltageMeasurement=phase-to-ground  SetLabelV=on  LabelV=V832  Vpu=off  VpuLL=off  CurrentMeasurement=no  SetLabelI=off  LabelI=I815  Ipu=off  Pbase=100e6  Vbase=24900  OutputType=Complex  PhasorSimulation=on  PSBequivalent=0
  832 D Z : Subsystem  mask(Three Phase Delta ZIP Load (Phasor)){Vnom=24900, fnom=60, Pnom=[7 2 6]*1e3/2 *a, Qnom=[3 1 3]*1e3/2*a, LoadType=Constant Z, Vlim=0.7}
      mask prompts: Vnom "Nominal Ph-Ph Voltage (Vrms)"; fnom "Nominal Frequency fn (Hz)"; Pnom "Nominal Per Phase Active Power [Pab Pbc Pca] (W)"; Qnom "Nominal Per Phase Reactive Power [Qab Qbc Qca] (VAR)"; LoadType "Load Type"; Vlim "Minimum Voltage (pu)"
      mask help:
      | Notes:
      | Three Phase Delta Connected ZIP load model which gets converted to constant Z type if the voltage becomes lower than the Minimum Voltage.
      mask TypeOptions LoadType: Constant Z | Constant I | Constant P
      mask DialogControl ParameterTabVar0 Prompt: Parameters
      mask DialogControl ParameterTabVar01 Prompt: Type
      mask Display:
      | color('red');
      | %load figure 0deg
      | A=[-210,-180,-170,-160,-147,-140,-130,-120,-110,-80,-50,-49,-45,-39,-33,-26,-21,-18,-17,-19,-22,-22,-26,-27,-25,-22,-16,-9,-3,2,6,6,4,1,1,-3,-4,-2,2,7,14,20,26,29,30,28,24,24,21,20,21,25,31,37,44,49,50,50,80];
      | B=[-41.5,-41.5,-63,-20,-63,-20,-63,-20,-41.5,-41.5,-41.5,-34,-26,-21,-20,-22,-28,-37,-47,-57,-63,-63,-54,-44,-34,-26,-21,-20,-22,-28,-37,-47,-57,-63,-63,-54,-44,-34,-26,-21,-20,-22,-28,-37,-47,-57,-63,-63,-54,-44,-34,-26,-21,-20,-22,-28,-37,-41.50,-41.5];
      | plot(A,B);
      | 
      | %load figure 0deg inverted
      | A1=[-80,-50,-49,-45,-39,-33,-26,-21,-18,-17,-19,-22,-22,-26,-27,-25,-22,-16,-9,-3,2,6,6,4,1,1,-3,-4,-2,2,7,14,20,26,29,30,28,24,24,21,20,21,25,31,37,44,49,50,50,80,110,120,130,143,150,160,170,180,210];
      | B1=[-41.5,-41.5,-34,-26,-21,-20,-22,-28,-37,-47,-57,-63,-63,-54,-44,-34,-26,-21,-20,-22,-28,-37,-47,-57,-63,-63,-54,-44,-34,-26,-21,-20,-22,-28,-37,-47,-57,-63,-63,-54,-44,-34,-26,-21,-20,-22,-28,-37,-41.5,-41.5,-41.5,-63,-20,-63,-20,-63,-20,-41.5,-41.5];
      | 
      | 
      | %load figure -120deg
      | c=1*exp(sqrt(-1)*(-60*pi/180));
      | l=A1+j*B1;
      | m=l*c;
      | E=real(m);F=imag(m);
      | E=E+10.94;F=F+161.1;
      | plot(E,F);
      | 
      | %load figure +120deg
      | c=1*exp(sqrt(-1)*(60*pi/180));
      | l=A1+j*B1;
      | m=l*c;
      | G=real(m);
      | H=imag(m);
      | G=G-205.94;H=H+48.53;
      | plot(G,H);
      | 
      | color('black');
      | port_label('LConn', 1, 'A')
      | port_label('LConn', 2, 'B')
      | port_label('LConn', 3, 'C')
  832-858 301 : spsThreePhasePISectionLineLib/Three-Phase PI Section Line  LConnTagsString=a|b|c  RConnTagsString=A|B|C  Length=4900*ft2km  Frequency=60  Resistances=[R1_301 R0_301]  Inductances=[L1_301 L0_301]  Capacitances=[C1_301 C0_301]
  834 : spsThreePhaseVIMeasurementLib/Three-Phase V-I Measurement  VoltageMeasurement=phase-to-ground  SetLabelV=on  LabelV=V834  Vpu=off  VpuLL=off  CurrentMeasurement=yes  SetLabelI=on  LabelI=I834  Ipu=off  Pbase=100e6  Vbase=24900  OutputType=Complex  PhasorSimulation=on  PSBequivalent=0
  834 D PQ : Subsystem  mask(Three Phase Delta ZIP Load (Phasor)){Vnom=24900, fnom=60, Pnom=[4 15 13]*1e3/2 *a, Qnom=[2 8 7]*1e3/2 *a, LoadType=Constant P, Vlim=0.7}
      mask prompts: Vnom "Nominal Ph-Ph Voltage (Vrms)"; fnom "Nominal Frequency fn (Hz)"; Pnom "Nominal Per Phase Active Power [Pab Pbc Pca] (W)"; Qnom "Nominal Per Phase Reactive Power [Qab Qbc Qca] (VAR)"; LoadType "Load Type"; Vlim "Minimum Voltage (pu)"
      mask help:
      | Notes:
      | Three Phase Delta Connected ZIP load model which gets converted to constant Z type if the voltage becomes lower than the Minimum Voltage.
      mask TypeOptions LoadType: Constant Z | Constant I | Constant P
      mask DialogControl ParameterTabVar0 Prompt: Parameters
      mask DialogControl ParameterTabVar01 Prompt: Type
      mask Display:
      | color('red');
      | %load figure 0deg
      | A=[-210,-180,-170,-160,-147,-140,-130,-120,-110,-80,-50,-49,-45,-39,-33,-26,-21,-18,-17,-19,-22,-22,-26,-27,-25,-22,-16,-9,-3,2,6,6,4,1,1,-3,-4,-2,2,7,14,20,26,29,30,28,24,24,21,20,21,25,31,37,44,49,50,50,80];
      | B=[-41.5,-41.5,-63,-20,-63,-20,-63,-20,-41.5,-41.5,-41.5,-34,-26,-21,-20,-22,-28,-37,-47,-57,-63,-63,-54,-44,-34,-26,-21,-20,-22,-28,-37,-47,-57,-63,-63,-54,-44,-34,-26,-21,-20,-22,-28,-37,-47,-57,-63,-63,-54,-44,-34,-26,-21,-20,-22,-28,-37,-41.50,-41.5];
      | plot(A,B);
      | 
      | %load figure 0deg inverted
      | A1=[-80,-50,-49,-45,-39,-33,-26,-21,-18,-17,-19,-22,-22,-26,-27,-25,-22,-16,-9,-3,2,6,6,4,1,1,-3,-4,-2,2,7,14,20,26,29,30,28,24,24,21,20,21,25,31,37,44,49,50,50,80,110,120,130,143,150,160,170,180,210];
      | B1=[-41.5,-41.5,-34,-26,-21,-20,-22,-28,-37,-47,-57,-63,-63,-54,-44,-34,-26,-21,-20,-22,-28,-37,-47,-57,-63,-63,-54,-44,-34,-26,-21,-20,-22,-28,-37,-47,-57,-63,-63,-54,-44,-34,-26,-21,-20,-22,-28,-37,-41.5,-41.5,-41.5,-63,-20,-63,-20,-63,-20,-41.5,-41.5];
      | 
      | 
      | %load figure -120deg
      | c=1*exp(sqrt(-1)*(-60*pi/180));
      | l=A1+j*B1;
      | m=l*c;
      | E=real(m);F=imag(m);
      | E=E+10.94;F=F+161.1;
      | plot(E,F);
      | 
      | %load figure +120deg
      | c=1*exp(sqrt(-1)*(60*pi/180));
      | l=A1+j*B1;
      | m=l*c;
      | G=real(m);
      | H=imag(m);
      | G=G-205.94;H=H+48.53;
      | plot(G,H);
      | 
      | color('black');
      | port_label('LConn', 1, 'A')
      | port_label('LConn', 2, 'B')
      | port_label('LConn', 3, 'C')
  834 D Z : Subsystem  mask(Three Phase Delta ZIP Load (Phasor)){Vnom=24900, fnom=60, Pnom=[16 20 110]*1e3/2 *a, Qnom=[8 10 55]*1e3/2*a, LoadType=Constant Z, Vlim=0.7}
      mask prompts: Vnom "Nominal Ph-Ph Voltage (Vrms)"; fnom "Nominal Frequency fn (Hz)"; Pnom "Nominal Per Phase Active Power [Pab Pbc Pca] (W)"; Qnom "Nominal Per Phase Reactive Power [Qab Qbc Qca] (VAR)"; LoadType "Load Type"; Vlim "Minimum Voltage (pu)"
      mask help:
      | Notes:
      | Three Phase Delta Connected ZIP load model which gets converted to constant Z type if the voltage becomes lower than the Minimum Voltage.
      mask TypeOptions LoadType: Constant Z | Constant I | Constant P
      mask DialogControl ParameterTabVar0 Prompt: Parameters
      mask DialogControl ParameterTabVar01 Prompt: Type
      mask Display:
      | color('red');
      | %load figure 0deg
      | A=[-210,-180,-170,-160,-147,-140,-130,-120,-110,-80,-50,-49,-45,-39,-33,-26,-21,-18,-17,-19,-22,-22,-26,-27,-25,-22,-16,-9,-3,2,6,6,4,1,1,-3,-4,-2,2,7,14,20,26,29,30,28,24,24,21,20,21,25,31,37,44,49,50,50,80];
      | B=[-41.5,-41.5,-63,-20,-63,-20,-63,-20,-41.5,-41.5,-41.5,-34,-26,-21,-20,-22,-28,-37,-47,-57,-63,-63,-54,-44,-34,-26,-21,-20,-22,-28,-37,-47,-57,-63,-63,-54,-44,-34,-26,-21,-20,-22,-28,-37,-47,-57,-63,-63,-54,-44,-34,-26,-21,-20,-22,-28,-37,-41.50,-41.5];
      | plot(A,B);
      | 
      | %load figure 0deg inverted
      | A1=[-80,-50,-49,-45,-39,-33,-26,-21,-18,-17,-19,-22,-22,-26,-27,-25,-22,-16,-9,-3,2,6,6,4,1,1,-3,-4,-2,2,7,14,20,26,29,30,28,24,24,21,20,21,25,31,37,44,49,50,50,80,110,120,130,143,150,160,170,180,210];
      | B1=[-41.5,-41.5,-34,-26,-21,-20,-22,-28,-37,-47,-57,-63,-63,-54,-44,-34,-26,-21,-20,-22,-28,-37,-47,-57,-63,-63,-54,-44,-34,-26,-21,-20,-22,-28,-37,-47,-57,-63,-63,-54,-44,-34,-26,-21,-20,-22,-28,-37,-41.5,-41.5,-41.5,-63,-20,-63,-20,-63,-20,-41.5,-41.5];
      | 
      | 
      | %load figure -120deg
      | c=1*exp(sqrt(-1)*(-60*pi/180));
      | l=A1+j*B1;
      | m=l*c;
      | E=real(m);F=imag(m);
      | E=E+10.94;F=F+161.1;
      | plot(E,F);
      | 
      | %load figure +120deg
      | c=1*exp(sqrt(-1)*(60*pi/180));
      | l=A1+j*B1;
      | m=l*c;
      | G=real(m);
      | H=imag(m);
      | G=G-205.94;H=H+48.53;
      | plot(G,H);
      | 
      | color('black');
      | port_label('LConn', 1, 'A')
      | port_label('LConn', 2, 'B')
      | port_label('LConn', 3, 'C')
  834-842 301 : spsThreePhasePISectionLineLib/Three-Phase PI Section Line  LConnTagsString=a|b|c  RConnTagsString=A|B|C  Length=280*ft2km  Frequency=60  Resistances=[R1_301 R0_301]  Inductances=[L1_301 L0_301]  Capacitances=[C1_301 C0_301]
  834-860 301 : spsThreePhasePISectionLineLib/Three-Phase PI Section Line  LConnTagsString=a|b|c  RConnTagsString=A|B|C  Length=2020*ft2km  Frequency=60  Resistances=[R1_301 R0_301]  Inductances=[L1_301 L0_301]  Capacitances=[C1_301 C0_301]
  836 : spsThreePhaseVIMeasurementLib/Three-Phase V-I Measurement  VoltageMeasurement=phase-to-ground  SetLabelV=on  LabelV=V836  Vpu=off  VpuLL=off  CurrentMeasurement=yes  SetLabelI=on  LabelI=I836  Ipu=off  Pbase=100e6  Vbase=24900  OutputType=Complex  PhasorSimulation=on  PSBequivalent=0
  836 D I : Subsystem  mask(Three Phase Delta ZIP Load (Phasor)){Vnom=24900, fnom=60, Pnom=[18 22 1e-3 ]*1e3/2 *a, Qnom=[9 11 0]*1e3/2 *a, LoadType=Constant I, Vlim=0.7}
      mask prompts: Vnom "Nominal Ph-Ph Voltage (Vrms)"; fnom "Nominal Frequency fn (Hz)"; Pnom "Nominal Per Phase Active Power [Pab Pbc Pca] (W)"; Qnom "Nominal Per Phase Reactive Power [Qab Qbc Qca] (VAR)"; LoadType "Load Type"; Vlim "Minimum Voltage (pu)"
      mask help:
      | Notes:
      | Three Phase Delta Connected ZIP load model which gets converted to constant Z type if the voltage becomes lower than the Minimum Voltage.
      mask TypeOptions LoadType: Constant Z | Constant I | Constant P
      mask DialogControl ParameterTabVar0 Prompt: Parameters
      mask DialogControl ParameterTabVar01 Prompt: Type
      mask Display:
      | color('red');
      | %load figure 0deg
      | A=[-210,-180,-170,-160,-147,-140,-130,-120,-110,-80,-50,-49,-45,-39,-33,-26,-21,-18,-17,-19,-22,-22,-26,-27,-25,-22,-16,-9,-3,2,6,6,4,1,1,-3,-4,-2,2,7,14,20,26,29,30,28,24,24,21,20,21,25,31,37,44,49,50,50,80];
      | B=[-41.5,-41.5,-63,-20,-63,-20,-63,-20,-41.5,-41.5,-41.5,-34,-26,-21,-20,-22,-28,-37,-47,-57,-63,-63,-54,-44,-34,-26,-21,-20,-22,-28,-37,-47,-57,-63,-63,-54,-44,-34,-26,-21,-20,-22,-28,-37,-47,-57,-63,-63,-54,-44,-34,-26,-21,-20,-22,-28,-37,-41.50,-41.5];
      | plot(A,B);
      | 
      | %load figure 0deg inverted
      | A1=[-80,-50,-49,-45,-39,-33,-26,-21,-18,-17,-19,-22,-22,-26,-27,-25,-22,-16,-9,-3,2,6,6,4,1,1,-3,-4,-2,2,7,14,20,26,29,30,28,24,24,21,20,21,25,31,37,44,49,50,50,80,110,120,130,143,150,160,170,180,210];
      | B1=[-41.5,-41.5,-34,-26,-21,-20,-22,-28,-37,-47,-57,-63,-63,-54,-44,-34,-26,-21,-20,-22,-28,-37,-47,-57,-63,-63,-54,-44,-34,-26,-21,-20,-22,-28,-37,-47,-57,-63,-63,-54,-44,-34,-26,-21,-20,-22,-28,-37,-41.5,-41.5,-41.5,-63,-20,-63,-20,-63,-20,-41.5,-41.5];
      | 
      | 
      | %load figure -120deg
      | c=1*exp(sqrt(-1)*(-60*pi/180));
      | l=A1+j*B1;
      | m=l*c;
      | E=real(m);F=imag(m);
      | E=E+10.94;F=F+161.1;
      | plot(E,F);
      | 
      | %load figure +120deg
      | c=1*exp(sqrt(-1)*(60*pi/180));
      | l=A1+j*B1;
      | m=l*c;
      | G=real(m);
      | H=imag(m);
      | G=G-205.94;H=H+48.53;
      | plot(G,H);
      | 
      | color('black');
      | port_label('LConn', 1, 'A')
      | port_label('LConn', 2, 'B')
      | port_label('LConn', 3, 'C')
  836 D PQ : Subsystem  mask(Three Phase Delta ZIP Load (Phasor)){Vnom=24900, fnom=60, Pnom=[30 10 42]*1e3/2 *a, Qnom=[15 6 22]*1e3/2 *a, LoadType=Constant P, Vlim=0.7}
      mask prompts: Vnom "Nominal Ph-Ph Voltage (Vrms)"; fnom "Nominal Frequency fn (Hz)"; Pnom "Nominal Per Phase Active Power [Pab Pbc Pca] (W)"; Qnom "Nominal Per Phase Reactive Power [Qab Qbc Qca] (VAR)"; LoadType "Load Type"; Vlim "Minimum Voltage (pu)"
      mask help:
      | Notes:
      | Three Phase Delta Connected ZIP load model which gets converted to constant Z type if the voltage becomes lower than the Minimum Voltage.
      mask TypeOptions LoadType: Constant Z | Constant I | Constant P
      mask DialogControl ParameterTabVar0 Prompt: Parameters
      mask DialogControl ParameterTabVar01 Prompt: Type
      mask Display:
      | color('red');
      | %load figure 0deg
      | A=[-210,-180,-170,-160,-147,-140,-130,-120,-110,-80,-50,-49,-45,-39,-33,-26,-21,-18,-17,-19,-22,-22,-26,-27,-25,-22,-16,-9,-3,2,6,6,4,1,1,-3,-4,-2,2,7,14,20,26,29,30,28,24,24,21,20,21,25,31,37,44,49,50,50,80];
      | B=[-41.5,-41.5,-63,-20,-63,-20,-63,-20,-41.5,-41.5,-41.5,-34,-26,-21,-20,-22,-28,-37,-47,-57,-63,-63,-54,-44,-34,-26,-21,-20,-22,-28,-37,-47,-57,-63,-63,-54,-44,-34,-26,-21,-20,-22,-28,-37,-47,-57,-63,-63,-54,-44,-34,-26,-21,-20,-22,-28,-37,-41.50,-41.5];
      | plot(A,B);
      | 
      | %load figure 0deg inverted
      | A1=[-80,-50,-49,-45,-39,-33,-26,-21,-18,-17,-19,-22,-22,-26,-27,-25,-22,-16,-9,-3,2,6,6,4,1,1,-3,-4,-2,2,7,14,20,26,29,30,28,24,24,21,20,21,25,31,37,44,49,50,50,80,110,120,130,143,150,160,170,180,210];
      | B1=[-41.5,-41.5,-34,-26,-21,-20,-22,-28,-37,-47,-57,-63,-63,-54,-44,-34,-26,-21,-20,-22,-28,-37,-47,-57,-63,-63,-54,-44,-34,-26,-21,-20,-22,-28,-37,-47,-57,-63,-63,-54,-44,-34,-26,-21,-20,-22,-28,-37,-41.5,-41.5,-41.5,-63,-20,-63,-20,-63,-20,-41.5,-41.5];
      | 
      | 
      | %load figure -120deg
      | c=1*exp(sqrt(-1)*(-60*pi/180));
      | l=A1+j*B1;
      | m=l*c;
      | E=real(m);F=imag(m);
      | E=E+10.94;F=F+161.1;
      | plot(E,F);
      | 
      | %load figure +120deg
      | c=1*exp(sqrt(-1)*(60*pi/180));
      | l=A1+j*B1;
      | m=l*c;
      | G=real(m);
      | H=imag(m);
      | G=G-205.94;H=H+48.53;
      | plot(G,H);
      | 
      | color('black');
      | port_label('LConn', 1, 'A')
      | port_label('LConn', 2, 'B')
      | port_label('LConn', 3, 'C')
  836-840 301 : spsThreePhasePISectionLineLib/Three-Phase PI Section Line  LConnTagsString=a|b|c  RConnTagsString=A|B|C  Length=860*ft2km  Frequency=60  Resistances=[R1_301 R0_301]  Inductances=[L1_301 L0_301]  Capacitances=[C1_301 C0_301]
  836-862 301 : spsThreePhasePISectionLineLib/Three-Phase PI Section Line  LConnTagsString=a|b|c  RConnTagsString=A|B|C  Length=280*ft2km  Frequency=60  Resistances=[R1_301 R0_301]  Inductances=[L1_301 L0_301]  Capacitances=[C1_301 C0_301]
  838 : Subsystem
  838 Y PQ : Subsystem  mask(Single Phase ZIP Load){Vnom=1.0*14376.02, fnom=60, Pnom=28e3/2 *a, Qnom=14e3/2*a, LoadType=constant P, Vlim=0.7}
      mask prompts: Vnom "Nominal Voltage Vn (Vrms)"; fnom "Nominal Frequency fn (Hz)"; Pnom "Nominal Active power (W)"; Qnom "Nominal Reactive power (VAR)"; LoadType "Load Type"; Vlim "Minimum voltage (pu)"
      mask help:
      | Notes:
      | Single Phase ZIP load model which gets converted to constant Z type if the voltage becomes lower than the Minimum Voltage.
      mask TypeOptions LoadType: Constant Z | constant I | constant P
      mask DialogControl ParameterTabVar0 Prompt: Parameters
      mask DialogControl ParameterTabVar1 Prompt: Type
      mask Display:
      | color('red');
      | A=[-210,-180,-170,-160,-147,-140,-130,-120,-110,-80,-50,-49,-45,-39,-33,-26,-21,-18,-17,-19,-22,-22,-26,-27,-25,-22,-16,-9,-3,2,6,6,4,1,1,-3,-4,-2,2,7,14,20,26,29,30,28,24,24,21,20,21,25,31,37,44,49,50,50,80];
      | B=[-41.5,-41.5,-63,-20,-63,-20,-63,-20,-41.5,-41.5,-41.5,-34,-26,-21,-20,-22,-28,-37,-47,-57,-63,-63,-54,-44,-34,-26,-21,-20,-22,-28,-37,-47,-57,-63,-63,-54,-44,-34,-26,-21,-20,-22,-28,-37,-47,-57,-63,-63,-54,-44,-34,-26,-21,-20,-22,-28,-37,-41.50,-41.5];
      | plot(A,B);
      | color('black');
      | port_label('LConn', 1, '+')
  840 : spsThreePhaseVIMeasurementLib/Three-Phase V-I Measurement  VoltageMeasurement=phase-to-ground  SetLabelV=on  LabelV=V840  Vpu=off  VpuLL=off  CurrentMeasurement=yes  SetLabelI=on  LabelI=I840  Ipu=off  Pbase=100e6  Vbase=24900  OutputType=Complex  PhasorSimulation=on  PSBequivalent=0
  840 D I : Subsystem  mask(Three Phase Delta ZIP Load (Phasor)){Vnom=24900, fnom=60, Pnom=[18 22 1e-3 ]*1e3/2 *a, Qnom=[9 11 0]*1e3/2 *a, LoadType=Constant I, Vlim=0.7}
      mask prompts: Vnom "Nominal Ph-Ph Voltage (Vrms)"; fnom "Nominal Frequency fn (Hz)"; Pnom "Nominal Per Phase Active Power [Pab Pbc Pca] (W)"; Qnom "Nominal Per Phase Reactive Power [Qab Qbc Qca] (VAR)"; LoadType "Load Type"; Vlim "Minimum Voltage (pu)"
      mask help:
      | Notes:
      | Three Phase Delta Connected ZIP load model which gets converted to constant Z type if the voltage becomes lower than the Minimum Voltage.
      mask TypeOptions LoadType: Constant Z | Constant I | Constant P
      mask DialogControl ParameterTabVar0 Prompt: Parameters
      mask DialogControl ParameterTabVar01 Prompt: Type
      mask Display:
      | color('red');
      | %load figure 0deg
      | A=[-210,-180,-170,-160,-147,-140,-130,-120,-110,-80,-50,-49,-45,-39,-33,-26,-21,-18,-17,-19,-22,-22,-26,-27,-25,-22,-16,-9,-3,2,6,6,4,1,1,-3,-4,-2,2,7,14,20,26,29,30,28,24,24,21,20,21,25,31,37,44,49,50,50,80];
      | B=[-41.5,-41.5,-63,-20,-63,-20,-63,-20,-41.5,-41.5,-41.5,-34,-26,-21,-20,-22,-28,-37,-47,-57,-63,-63,-54,-44,-34,-26,-21,-20,-22,-28,-37,-47,-57,-63,-63,-54,-44,-34,-26,-21,-20,-22,-28,-37,-47,-57,-63,-63,-54,-44,-34,-26,-21,-20,-22,-28,-37,-41.50,-41.5];
      | plot(A,B);
      | 
      | %load figure 0deg inverted
      | A1=[-80,-50,-49,-45,-39,-33,-26,-21,-18,-17,-19,-22,-22,-26,-27,-25,-22,-16,-9,-3,2,6,6,4,1,1,-3,-4,-2,2,7,14,20,26,29,30,28,24,24,21,20,21,25,31,37,44,49,50,50,80,110,120,130,143,150,160,170,180,210];
      | B1=[-41.5,-41.5,-34,-26,-21,-20,-22,-28,-37,-47,-57,-63,-63,-54,-44,-34,-26,-21,-20,-22,-28,-37,-47,-57,-63,-63,-54,-44,-34,-26,-21,-20,-22,-28,-37,-47,-57,-63,-63,-54,-44,-34,-26,-21,-20,-22,-28,-37,-41.5,-41.5,-41.5,-63,-20,-63,-20,-63,-20,-41.5,-41.5];
      | 
      | 
      | %load figure -120deg
      | c=1*exp(sqrt(-1)*(-60*pi/180));
      | l=A1+j*B1;
      | m=l*c;
      | E=real(m);F=imag(m);
      | E=E+10.94;F=F+161.1;
      | plot(E,F);
      | 
      | %load figure +120deg
      | c=1*exp(sqrt(-1)*(60*pi/180));
      | l=A1+j*B1;
      | m=l*c;
      | G=real(m);
      | H=imag(m);
      | G=G-205.94;H=H+48.53;
      | plot(G,H);
      | 
      | color('black');
      | port_label('LConn', 1, 'A')
      | port_label('LConn', 2, 'B')
      | port_label('LConn', 3, 'C')
  840 Y I : Subsystem  mask(Three Phase Star ZIP Load (Phasor)){Vnom=24900, fnom=60, Pnom=[9 9 9]*1e3 *a, Qnom=[7 7 7]*1e3*a, LoadType=Constant I, Vlim=0.7}
      mask prompts: Vnom "Nominal Ph-Ph voltage (Vrms)"; fnom "Nominal Frequency fn (Hz)"; Pnom "Nominal Per Phase Active Power [Pa Pb Pc] (W)"; Qnom "Nominal Per Phase Reactive Power [Qa Qb Qc] (VAR)"; LoadType "Load Type"; Vlim "Minimum voltage (pu)"
      mask help:
      | Notes:
      | Three Phase Star Connected ZIP load model which gets converted to constant Z type if the voltage becomes lower than the Minimum Voltage.
      mask TypeOptions LoadType: Constant Z | Constant I | Constant P
      mask DialogControl ParameterTabVar0 Prompt: Parameters
      mask DialogControl ParameterTabVar01 Prompt: Type
      mask Display:
      | color('red');
      | %load figure 0deg
      | A=[-210,-180,-170,-160,-147,-140,-130,-120,-110,-80,-50,-49,-45,-39,-33,-26,-21,-18,-17,-19,-22,-22,-26,-27,-25,-22,-16,-9,-3,2,6,6,4,1,1,-3,-4,-2,2,7,14,20,26,29,30,28,24,24,21,20,21,25,31,37,44,49,50,50,80];
      | B=[-41.5,-41.5,-63,-20,-63,-20,-63,-20,-41.5,-41.5,-41.5,-34,-26,-21,-20,-22,-28,-37,-47,-57,-63,-63,-54,-44,-34,-26,-21,-20,-22,-28,-37,-47,-57,-63,-63,-54,-44,-34,-26,-21,-20,-22,-28,-37,-47,-57,-63,-63,-54,-44,-34,-26,-21,-20,-22,-28,-37,-41.50,-41.5];
      | % plot(A,B);
      | 
      | %load figure 0deg inverted
      | A1=[-80,-50,-49,-45,-39,-33,-26,-21,-18,-17,-19,-22,-22,-26,-27,-25,-22,-16,-9,-3,2,6,6,4,1,1,-3,-4,-2,2,7,14,20,26,29,30,28,24,24,21,20,21,25,31,37,44,49,50,50,80,110,120,130,143,150,160,170,180,210];
      | B1=[-41.5,-41.5,-34,-26,-21,-20,-22,-28,-37,-47,-57,-63,-63,-54,-44,-34,-26,-21,-20,-22,-28,-37,-47,-57,-63,-63,-54,-44,-34,-26,-21,-20,-22,-28,-37,-47,-57,-63,-63,-54,-44,-34,-26,-21,-20,-22,-28,-37,-41.5,-41.5,-41.5,-63,-20,-63,-20,-63,-20,-41.5,-41.5];
      | 
      | 
      | %load figure 90deg
      | C=[-41.5,-41.5,-20,-63,-20,-63,-20,-63,-41.5,-41.5,-41.5,-37,-28,-22,-20,-21,-26,-34,-44,-54,-63,-63,-57,-47,-37,-28,-22,-20,-21,-26,-34,-44,-54,-63,-63,-57,-47,-37,-28,-22,-20,-21,-26,-34,-44,-54,-63,-63,-57,-47,-37,-28,-22,-20,-21,-26,-34,-41.5,-41.5];
      | D=[190,160,150,140,130,123,110,100,90,80,50,50,49,44,37,31,25,21,20,21,24,24,28,30,29,26,20,14,7,2,-2,-4,-3,1,1,4,6,6,2,-3,-9,-16,-22,-25,-27,-26,-22,-22,-19,-17,-18,-21,-26,-33,-39,-45,-49,-50,-70];
      | plot(C,D);
      | 
      | 
      | %load figure -120deg
      | c=1*exp(sqrt(-1)*(-60*pi/180));
      | l=A1+j*B1;
      | m=l*c;
      | E=real(m);F=imag(m);
      | E=E+34.4400;F=F-118.53;
      | plot(E,F);
      | 
      | %load figure +120deg
      | c=1*exp(sqrt(-1)*(60*pi/180));
      | l=A+j*B;
      | m=l*c;
      | G=real(m);
      | H=imag(m);
      | G=G-117.44;H=H-118.5300;
      | plot(G,H);
      | 
      | color('black');
      | port_label('LConn', 1, 'A')
      | port_label('LConn', 2, 'B')
      | port_label('LConn', 3, 'C')
  842 : spsThreePhaseVIMeasurementLib/Three-Phase V-I Measurement  VoltageMeasurement=phase-to-ground  SetLabelV=on  LabelV=V842  Vpu=off  VpuLL=off  CurrentMeasurement=yes  SetLabelI=on  LabelI=I842  Ipu=off  Pbase=100e6  Vbase=24900  OutputType=Complex  PhasorSimulation=on  PSBequivalent=0
  842 Y PQ : Subsystem  mask(Single Phase ZIP Load){Vnom=1.0*14376.02, fnom=60, Pnom=9e3/2 *a, Qnom=5e3/2 *a, LoadType=constant P, Vlim=0.7}
      mask prompts: Vnom "Nominal Voltage Vn (Vrms)"; fnom "Nominal Frequency fn (Hz)"; Pnom "Nominal Active power (W)"; Qnom "Nominal Reactive power (VAR)"; LoadType "Load Type"; Vlim "Minimum voltage (pu)"
      mask help:
      | Notes:
      | Single Phase ZIP load model which gets converted to constant Z type if the voltage becomes lower than the Minimum Voltage.
      mask TypeOptions LoadType: Constant Z | constant I | constant P
      mask DialogControl ParameterTabVar0 Prompt: Parameters
      mask DialogControl ParameterTabVar1 Prompt: Type
      mask Display:
      | color('red');
      | A=[-210,-180,-170,-160,-147,-140,-130,-120,-110,-80,-50,-49,-45,-39,-33,-26,-21,-18,-17,-19,-22,-22,-26,-27,-25,-22,-16,-9,-3,2,6,6,4,1,1,-3,-4,-2,2,7,14,20,26,29,30,28,24,24,21,20,21,25,31,37,44,49,50,50,80];
      | B=[-41.5,-41.5,-63,-20,-63,-20,-63,-20,-41.5,-41.5,-41.5,-34,-26,-21,-20,-22,-28,-37,-47,-57,-63,-63,-54,-44,-34,-26,-21,-20,-22,-28,-37,-47,-57,-63,-63,-54,-44,-34,-26,-21,-20,-22,-28,-37,-47,-57,-63,-63,-54,-44,-34,-26,-21,-20,-22,-28,-37,-41.50,-41.5];
      | plot(A,B);
      | color('black');
      | port_label('LConn', 1, '+')
  842-844 301 : spsThreePhasePISectionLineLib/Three-Phase PI Section Line  LConnTagsString=a|b|c  RConnTagsString=A|B|C  Length=1350*ft2km  Frequency=60  Resistances=[R1_301 R0_301]  Inductances=[L1_301 L0_301]  Capacitances=[C1_301 C0_301]
  844 : spsThreePhaseVIMeasurementLib/Three-Phase V-I Measurement  VoltageMeasurement=phase-to-ground  SetLabelV=on  LabelV=V844  Vpu=off  VpuLL=off  CurrentMeasurement=yes  SetLabelI=on  LabelI=I844  Ipu=off  Pbase=100e6  Vbase=24900  OutputType=Complex  PhasorSimulation=on  PSBequivalent=0
  844 Y PQ : Subsystem  mask(Single Phase ZIP Load){Vnom=1.0*14376.02, fnom=60, Pnom=9*1e3/2 *a, Qnom=5*1e3/2 *a, LoadType=constant P, Vlim=0.7}
      mask prompts: Vnom "Nominal Voltage Vn (Vrms)"; fnom "Nominal Frequency fn (Hz)"; Pnom "Nominal Active power (W)"; Qnom "Nominal Reactive power (VAR)"; LoadType "Load Type"; Vlim "Minimum voltage (pu)"
      mask help:
      | Notes:
      | Single Phase ZIP load model which gets converted to constant Z type if the voltage becomes lower than the Minimum Voltage.
      mask TypeOptions LoadType: Constant Z | constant I | constant P
      mask DialogControl ParameterTabVar0 Prompt: Parameters
      mask DialogControl ParameterTabVar1 Prompt: Type
      mask Display:
      | color('red');
      | A=[-210,-180,-170,-160,-147,-140,-130,-120,-110,-80,-50,-49,-45,-39,-33,-26,-21,-18,-17,-19,-22,-22,-26,-27,-25,-22,-16,-9,-3,2,6,6,4,1,1,-3,-4,-2,2,7,14,20,26,29,30,28,24,24,21,20,21,25,31,37,44,49,50,50,80];
      | B=[-41.5,-41.5,-63,-20,-63,-20,-63,-20,-41.5,-41.5,-41.5,-34,-26,-21,-20,-22,-28,-37,-47,-57,-63,-63,-54,-44,-34,-26,-21,-20,-22,-28,-37,-47,-57,-63,-63,-54,-44,-34,-26,-21,-20,-22,-28,-37,-47,-57,-63,-63,-54,-44,-34,-26,-21,-20,-22,-28,-37,-41.50,-41.5];
      | plot(A,B);
      | color('black');
      | port_label('LConn', 1, '+')
  844 Y PQ1 : Subsystem  mask(Three Phase Star ZIP Load (Phasor)){Vnom=24900, fnom=60, Pnom=[1e-3  25 20]*1e3/2 *a, Qnom=[0 12 11]*1e3/2*a, LoadType=Constant P, Vlim=0.7}
      mask prompts: Vnom "Nominal Ph-Ph voltage (Vrms)"; fnom "Nominal Frequency fn (Hz)"; Pnom "Nominal Per Phase Active Power [Pa Pb Pc] (W)"; Qnom "Nominal Per Phase Reactive Power [Qa Qb Qc] (VAR)"; LoadType "Load Type"; Vlim "Minimum voltage (pu)"
      mask help:
      | Notes:
      | Three Phase Star Connected ZIP load model which gets converted to constant Z type if the voltage becomes lower than the Minimum Voltage.
      mask TypeOptions LoadType: Constant Z | Constant I | Constant P
      mask DialogControl ParameterTabVar0 Prompt: Parameters
      mask DialogControl ParameterTabVar01 Prompt: Type
      mask Display:
      | color('red');
      | %load figure 0deg
      | A=[-210,-180,-170,-160,-147,-140,-130,-120,-110,-80,-50,-49,-45,-39,-33,-26,-21,-18,-17,-19,-22,-22,-26,-27,-25,-22,-16,-9,-3,2,6,6,4,1,1,-3,-4,-2,2,7,14,20,26,29,30,28,24,24,21,20,21,25,31,37,44,49,50,50,80];
      | B=[-41.5,-41.5,-63,-20,-63,-20,-63,-20,-41.5,-41.5,-41.5,-34,-26,-21,-20,-22,-28,-37,-47,-57,-63,-63,-54,-44,-34,-26,-21,-20,-22,-28,-37,-47,-57,-63,-63,-54,-44,-34,-26,-21,-20,-22,-28,-37,-47,-57,-63,-63,-54,-44,-34,-26,-21,-20,-22,-28,-37,-41.50,-41.5];
      | % plot(A,B);
      | 
      | %load figure 0deg inverted
      | A1=[-80,-50,-49,-45,-39,-33,-26,-21,-18,-17,-19,-22,-22,-26,-27,-25,-22,-16,-9,-3,2,6,6,4,1,1,-3,-4,-2,2,7,14,20,26,29,30,28,24,24,21,20,21,25,31,37,44,49,50,50,80,110,120,130,143,150,160,170,180,210];
      | B1=[-41.5,-41.5,-34,-26,-21,-20,-22,-28,-37,-47,-57,-63,-63,-54,-44,-34,-26,-21,-20,-22,-28,-37,-47,-57,-63,-63,-54,-44,-34,-26,-21,-20,-22,-28,-37,-47,-57,-63,-63,-54,-44,-34,-26,-21,-20,-22,-28,-37,-41.5,-41.5,-41.5,-63,-20,-63,-20,-63,-20,-41.5,-41.5];
      | 
      | 
      | %load figure 90deg
      | C=[-41.5,-41.5,-20,-63,-20,-63,-20,-63,-41.5,-41.5,-41.5,-37,-28,-22,-20,-21,-26,-34,-44,-54,-63,-63,-57,-47,-37,-28,-22,-20,-21,-26,-34,-44,-54,-63,-63,-57,-47,-37,-28,-22,-20,-21,-26,-34,-44,-54,-63,-63,-57,-47,-37,-28,-22,-20,-21,-26,-34,-41.5,-41.5];
      | D=[190,160,150,140,130,123,110,100,90,80,50,50,49,44,37,31,25,21,20,21,24,24,28,30,29,26,20,14,7,2,-2,-4,-3,1,1,4,6,6,2,-3,-9,-16,-22,-25,-27,-26,-22,-22,-19,-17,-18,-21,-26,-33,-39,-45,-49,-50,-70];
      | plot(C,D);
      | 
      | 
      | %load figure -120deg
      | c=1*exp(sqrt(-1)*(-60*pi/180));
      | l=A1+j*B1;
      | m=l*c;
      | E=real(m);F=imag(m);
      | E=E+34.4400;F=F-118.53;
      | plot(E,F);
      | 
      | %load figure +120deg
      | c=1*exp(sqrt(-1)*(60*pi/180));
      | l=A+j*B;
      | m=l*c;
      | G=real(m);
      | H=imag(m);
      | G=G-117.44;H=H-118.5300;
      | plot(G,H);
      | 
      | color('black');
      | port_label('LConn', 1, 'A')
      | port_label('LConn', 2, 'B')
      | port_label('LConn', 3, 'C')
  844 Y Z : Subsystem  mask(Three Phase Star ZIP Load (Phasor)){Vnom=24900, fnom=60, Pnom=[135 135 135]*1e3 *a, Qnom=[105 105 105]*1e3*a, LoadType=Constant Z, Vlim=0.7}
      mask prompts: Vnom "Nominal Ph-Ph voltage (Vrms)"; fnom "Nominal Frequency fn (Hz)"; Pnom "Nominal Per Phase Active Power [Pa Pb Pc] (W)"; Qnom "Nominal Per Phase Reactive Power [Qa Qb Qc] (VAR)"; LoadType "Load Type"; Vlim "Minimum voltage (pu)"
      mask help:
      | Notes:
      | Three Phase Star Connected ZIP load model which gets converted to constant Z type if the voltage becomes lower than the Minimum Voltage.
      mask TypeOptions LoadType: Constant Z | Constant I | Constant P
      mask DialogControl ParameterTabVar0 Prompt: Parameters
      mask DialogControl ParameterTabVar01 Prompt: Type
      mask Display:
      | color('red');
      | %load figure 0deg
      | A=[-210,-180,-170,-160,-147,-140,-130,-120,-110,-80,-50,-49,-45,-39,-33,-26,-21,-18,-17,-19,-22,-22,-26,-27,-25,-22,-16,-9,-3,2,6,6,4,1,1,-3,-4,-2,2,7,14,20,26,29,30,28,24,24,21,20,21,25,31,37,44,49,50,50,80];
      | B=[-41.5,-41.5,-63,-20,-63,-20,-63,-20,-41.5,-41.5,-41.5,-34,-26,-21,-20,-22,-28,-37,-47,-57,-63,-63,-54,-44,-34,-26,-21,-20,-22,-28,-37,-47,-57,-63,-63,-54,-44,-34,-26,-21,-20,-22,-28,-37,-47,-57,-63,-63,-54,-44,-34,-26,-21,-20,-22,-28,-37,-41.50,-41.5];
      | % plot(A,B);
      | 
      | %load figure 0deg inverted
      | A1=[-80,-50,-49,-45,-39,-33,-26,-21,-18,-17,-19,-22,-22,-26,-27,-25,-22,-16,-9,-3,2,6,6,4,1,1,-3,-4,-2,2,7,14,20,26,29,30,28,24,24,21,20,21,25,31,37,44,49,50,50,80,110,120,130,143,150,160,170,180,210];
      | B1=[-41.5,-41.5,-34,-26,-21,-20,-22,-28,-37,-47,-57,-63,-63,-54,-44,-34,-26,-21,-20,-22,-28,-37,-47,-57,-63,-63,-54,-44,-34,-26,-21,-20,-22,-28,-37,-47,-57,-63,-63,-54,-44,-34,-26,-21,-20,-22,-28,-37,-41.5,-41.5,-41.5,-63,-20,-63,-20,-63,-20,-41.5,-41.5];
      | 
      | 
      | %load figure 90deg
      | C=[-41.5,-41.5,-20,-63,-20,-63,-20,-63,-41.5,-41.5,-41.5,-37,-28,-22,-20,-21,-26,-34,-44,-54,-63,-63,-57,-47,-37,-28,-22,-20,-21,-26,-34,-44,-54,-63,-63,-57,-47,-37,-28,-22,-20,-21,-26,-34,-44,-54,-63,-63,-57,-47,-37,-28,-22,-20,-21,-26,-34,-41.5,-41.5];
      | D=[190,160,150,140,130,123,110,100,90,80,50,50,49,44,37,31,25,21,20,21,24,24,28,30,29,26,20,14,7,2,-2,-4,-3,1,1,4,6,6,2,-3,-9,-16,-22,-25,-27,-26,-22,-22,-19,-17,-18,-21,-26,-33,-39,-45,-49,-50,-70];
      | plot(C,D);
      | 
      | 
      | %load figure -120deg
      | c=1*exp(sqrt(-1)*(-60*pi/180));
      | l=A1+j*B1;
      | m=l*c;
      | E=real(m);F=imag(m);
      | E=E+34.4400;F=F-118.53;
      | plot(E,F);
      | 
      | %load figure +120deg
      | c=1*exp(sqrt(-1)*(60*pi/180));
      | l=A+j*B;
      | m=l*c;
      | G=real(m);
      | H=imag(m);
      | G=G-117.44;H=H-118.5300;
      | plot(G,H);
      | 
      | color('black');
      | port_label('LConn', 1, 'A')
      | port_label('LConn', 2, 'B')
      | port_label('LConn', 3, 'C')
  844 Yg Z : spsThreePhaseSeriesRLCLoadLib/Three-Phase Series RLC Load  LConnTagsString=A|B|C  Configuration=Y (grounded)  NominalVoltage=1000  Vabc=[ 1.0 1.0 1.0]*14376.02  Vabcp=[1e3 1e3 1e3]  NominalFrequency=60  UnbalancedPower=on  ActivePower=0  InductivePower=0  CapacitivePower=100  Pabc=[0 0 0]  QLabc=[0 0 0]  QCabc=[100 100 100]*1e3*a  Pabcp=[10e3 9e3 11e3]  QLabcp=[100 90 110]  QCabcp=[100 90 110]  Measurements=None  LoadType=constant Z
  844-846 301 : spsThreePhasePISectionLineLib/Three-Phase PI Section Line  LConnTagsString=a|b|c  RConnTagsString=A|B|C  Length=3640*ft2km  Frequency=60  Resistances=[R1_301 R0_301]  Inductances=[L1_301 L0_301]  Capacitances=[C1_301 C0_301]
  846 : spsThreePhaseVIMeasurementLib/Three-Phase V-I Measurement  VoltageMeasurement=phase-to-ground  SetLabelV=on  LabelV=V846  Vpu=off  VpuLL=off  CurrentMeasurement=yes  SetLabelI=on  LabelI=I846  Ipu=off  Pbase=100e6  Vbase=24900  OutputType=Complex  PhasorSimulation=on  PSBequivalent=0
  846 Y PQ : Subsystem  mask(Three Phase Star ZIP Load (Phasor)){Vnom=24900, fnom=60, Pnom=[1e-3  25 20]*1e3/2 *a, Qnom=[0 12 11]*1e3/2*a, LoadType=Constant P, Vlim=0.7}
      mask prompts: Vnom "Nominal Ph-Ph voltage (Vrms)"; fnom "Nominal Frequency fn (Hz)"; Pnom "Nominal Per Phase Active Power [Pa Pb Pc] (W)"; Qnom "Nominal Per Phase Reactive Power [Qa Qb Qc] (VAR)"; LoadType "Load Type"; Vlim "Minimum voltage (pu)"
      mask help:
      | Notes:
      | Three Phase Star Connected ZIP load model which gets converted to constant Z type if the voltage becomes lower than the Minimum Voltage.
      mask TypeOptions LoadType: Constant Z | Constant I | Constant P
      mask DialogControl ParameterTabVar0 Prompt: Parameters
      mask DialogControl ParameterTabVar01 Prompt: Type
      mask Display:
      | color('red');
      | %load figure 0deg
      | A=[-210,-180,-170,-160,-147,-140,-130,-120,-110,-80,-50,-49,-45,-39,-33,-26,-21,-18,-17,-19,-22,-22,-26,-27,-25,-22,-16,-9,-3,2,6,6,4,1,1,-3,-4,-2,2,7,14,20,26,29,30,28,24,24,21,20,21,25,31,37,44,49,50,50,80];
      | B=[-41.5,-41.5,-63,-20,-63,-20,-63,-20,-41.5,-41.5,-41.5,-34,-26,-21,-20,-22,-28,-37,-47,-57,-63,-63,-54,-44,-34,-26,-21,-20,-22,-28,-37,-47,-57,-63,-63,-54,-44,-34,-26,-21,-20,-22,-28,-37,-47,-57,-63,-63,-54,-44,-34,-26,-21,-20,-22,-28,-37,-41.50,-41.5];
      | % plot(A,B);
      | 
      | %load figure 0deg inverted
      | A1=[-80,-50,-49,-45,-39,-33,-26,-21,-18,-17,-19,-22,-22,-26,-27,-25,-22,-16,-9,-3,2,6,6,4,1,1,-3,-4,-2,2,7,14,20,26,29,30,28,24,24,21,20,21,25,31,37,44,49,50,50,80,110,120,130,143,150,160,170,180,210];
      | B1=[-41.5,-41.5,-34,-26,-21,-20,-22,-28,-37,-47,-57,-63,-63,-54,-44,-34,-26,-21,-20,-22,-28,-37,-47,-57,-63,-63,-54,-44,-34,-26,-21,-20,-22,-28,-37,-47,-57,-63,-63,-54,-44,-34,-26,-21,-20,-22,-28,-37,-41.5,-41.5,-41.5,-63,-20,-63,-20,-63,-20,-41.5,-41.5];
      | 
      | 
      | %load figure 90deg
      | C=[-41.5,-41.5,-20,-63,-20,-63,-20,-63,-41.5,-41.5,-41.5,-37,-28,-22,-20,-21,-26,-34,-44,-54,-63,-63,-57,-47,-37,-28,-22,-20,-21,-26,-34,-44,-54,-63,-63,-57,-47,-37,-28,-22,-20,-21,-26,-34,-44,-54,-63,-63,-57,-47,-37,-28,-22,-20,-21,-26,-34,-41.5,-41.5];
      | D=[190,160,150,140,130,123,110,100,90,80,50,50,49,44,37,31,25,21,20,21,24,24,28,30,29,26,20,14,7,2,-2,-4,-3,1,1,4,6,6,2,-3,-9,-16,-22,-25,-27,-26,-22,-22,-19,-17,-18,-21,-26,-33,-39,-45,-49,-50,-70];
      | plot(C,D);
      | 
      | 
      | %load figure -120deg
      | c=1*exp(sqrt(-1)*(-60*pi/180));
      | l=A1+j*B1;
      | m=l*c;
      | E=real(m);F=imag(m);
      | E=E+34.4400;F=F-118.53;
      | plot(E,F);
      | 
      | %load figure +120deg
      | c=1*exp(sqrt(-1)*(60*pi/180));
      | l=A+j*B;
      | m=l*c;
      | G=real(m);
      | H=imag(m);
      | G=G-117.44;H=H-118.5300;
      | plot(G,H);
      | 
      | color('black');
      | port_label('LConn', 1, 'A')
      | port_label('LConn', 2, 'B')
      | port_label('LConn', 3, 'C')
  846 Y PQ1 : Subsystem  mask(Single Phase ZIP Load){Vnom=1.0*14376.02, fnom=60, Pnom=23e3/2 *a, Qnom=11e3/2 *a, LoadType=constant P, Vlim=0.7}
      mask prompts: Vnom "Nominal Voltage Vn (Vrms)"; fnom "Nominal Frequency fn (Hz)"; Pnom "Nominal Active power (W)"; Qnom "Nominal Reactive power (VAR)"; LoadType "Load Type"; Vlim "Minimum voltage (pu)"
      mask help:
      | Notes:
      | Single Phase ZIP load model which gets converted to constant Z type if the voltage becomes lower than the Minimum Voltage.
      mask TypeOptions LoadType: Constant Z | constant I | constant P
      mask DialogControl ParameterTabVar0 Prompt: Parameters
      mask DialogControl ParameterTabVar1 Prompt: Type
      mask Display:
      | color('red');
      | A=[-210,-180,-170,-160,-147,-140,-130,-120,-110,-80,-50,-49,-45,-39,-33,-26,-21,-18,-17,-19,-22,-22,-26,-27,-25,-22,-16,-9,-3,2,6,6,4,1,1,-3,-4,-2,2,7,14,20,26,29,30,28,24,24,21,20,21,25,31,37,44,49,50,50,80];
      | B=[-41.5,-41.5,-63,-20,-63,-20,-63,-20,-41.5,-41.5,-41.5,-34,-26,-21,-20,-22,-28,-37,-47,-57,-63,-63,-54,-44,-34,-26,-21,-20,-22,-28,-37,-47,-57,-63,-63,-54,-44,-34,-26,-21,-20,-22,-28,-37,-47,-57,-63,-63,-54,-44,-34,-26,-21,-20,-22,-28,-37,-41.50,-41.5];
      | plot(A,B);
      | color('black');
      | port_label('LConn', 1, '+')
  846-848 301 : spsThreePhasePISectionLineLib/Three-Phase PI Section Line  LConnTagsString=a|b|c  RConnTagsString=A|B|C  Length=530*ft2km  Frequency=60  Resistances=[R1_301 R0_301]  Inductances=[L1_301 L0_301]  Capacitances=[C1_301 C0_301]
  "848 " : spsThreePhaseVIMeasurementLib/Three-Phase V-I Measurement  VoltageMeasurement=phase-to-ground  SetLabelV=on  LabelV=V848  Vpu=off  VpuLL=off  CurrentMeasurement=yes  SetLabelI=on  LabelI=I848  Ipu=off  Pbase=100e6  Vbase=24900  OutputType=Complex  PhasorSimulation=on  PSBequivalent=0
  848 D PQ : Subsystem  mask(Three Phase Delta ZIP Load (Phasor)){Vnom=24900, fnom=60, Pnom=[20 20 20]*1e3 *a, Qnom=[16 16 16]*1e3 *a, LoadType=Constant P, Vlim=0.7}
      mask prompts: Vnom "Nominal Ph-Ph Voltage (Vrms)"; fnom "Nominal Frequency fn (Hz)"; Pnom "Nominal Per Phase Active Power [Pab Pbc Pca] (W)"; Qnom "Nominal Per Phase Reactive Power [Qab Qbc Qca] (VAR)"; LoadType "Load Type"; Vlim "Minimum Voltage (pu)"
      mask help:
      | Notes:
      | Three Phase Delta Connected ZIP load model which gets converted to constant Z type if the voltage becomes lower than the Minimum Voltage.
      mask TypeOptions LoadType: Constant Z | Constant I | Constant P
      mask DialogControl ParameterTabVar0 Prompt: Parameters
      mask DialogControl ParameterTabVar01 Prompt: Type
      mask Display:
      | color('red');
      | %load figure 0deg
      | A=[-210,-180,-170,-160,-147,-140,-130,-120,-110,-80,-50,-49,-45,-39,-33,-26,-21,-18,-17,-19,-22,-22,-26,-27,-25,-22,-16,-9,-3,2,6,6,4,1,1,-3,-4,-2,2,7,14,20,26,29,30,28,24,24,21,20,21,25,31,37,44,49,50,50,80];
      | B=[-41.5,-41.5,-63,-20,-63,-20,-63,-20,-41.5,-41.5,-41.5,-34,-26,-21,-20,-22,-28,-37,-47,-57,-63,-63,-54,-44,-34,-26,-21,-20,-22,-28,-37,-47,-57,-63,-63,-54,-44,-34,-26,-21,-20,-22,-28,-37,-47,-57,-63,-63,-54,-44,-34,-26,-21,-20,-22,-28,-37,-41.50,-41.5];
      | plot(A,B);
      | 
      | %load figure 0deg inverted
      | A1=[-80,-50,-49,-45,-39,-33,-26,-21,-18,-17,-19,-22,-22,-26,-27,-25,-22,-16,-9,-3,2,6,6,4,1,1,-3,-4,-2,2,7,14,20,26,29,30,28,24,24,21,20,21,25,31,37,44,49,50,50,80,110,120,130,143,150,160,170,180,210];
      | B1=[-41.5,-41.5,-34,-26,-21,-20,-22,-28,-37,-47,-57,-63,-63,-54,-44,-34,-26,-21,-20,-22,-28,-37,-47,-57,-63,-63,-54,-44,-34,-26,-21,-20,-22,-28,-37,-47,-57,-63,-63,-54,-44,-34,-26,-21,-20,-22,-28,-37,-41.5,-41.5,-41.5,-63,-20,-63,-20,-63,-20,-41.5,-41.5];
      | 
      | 
      | %load figure -120deg
      | c=1*exp(sqrt(-1)*(-60*pi/180));
      | l=A1+j*B1;
      | m=l*c;
      | E=real(m);F=imag(m);
      | E=E+10.94;F=F+161.1;
      | plot(E,F);
      | 
      | %load figure +120deg
      | c=1*exp(sqrt(-1)*(60*pi/180));
      | l=A1+j*B1;
      | m=l*c;
      | G=real(m);
      | H=imag(m);
      | G=G-205.94;H=H+48.53;
      | plot(G,H);
      | 
      | color('black');
      | port_label('LConn', 1, 'A')
      | port_label('LConn', 2, 'B')
      | port_label('LConn', 3, 'C')
  848 Y PQ : Subsystem  mask(Single Phase ZIP Load){Vnom=1.0*14376.02, fnom=60, Pnom=23e3/2 *a, Qnom=11e3/2 *a, LoadType=constant P, Vlim=0.7}
      mask prompts: Vnom "Nominal Voltage Vn (Vrms)"; fnom "Nominal Frequency fn (Hz)"; Pnom "Nominal Active power (W)"; Qnom "Nominal Reactive power (VAR)"; LoadType "Load Type"; Vlim "Minimum voltage (pu)"
      mask help:
      | Notes:
      | Single Phase ZIP load model which gets converted to constant Z type if the voltage becomes lower than the Minimum Voltage.
      mask TypeOptions LoadType: Constant Z | constant I | constant P
      mask DialogControl ParameterTabVar0 Prompt: Parameters
      mask DialogControl ParameterTabVar1 Prompt: Type
      mask Display:
      | color('red');
      | A=[-210,-180,-170,-160,-147,-140,-130,-120,-110,-80,-50,-49,-45,-39,-33,-26,-21,-18,-17,-19,-22,-22,-26,-27,-25,-22,-16,-9,-3,2,6,6,4,1,1,-3,-4,-2,2,7,14,20,26,29,30,28,24,24,21,20,21,25,31,37,44,49,50,50,80];
      | B=[-41.5,-41.5,-63,-20,-63,-20,-63,-20,-41.5,-41.5,-41.5,-34,-26,-21,-20,-22,-28,-37,-47,-57,-63,-63,-54,-44,-34,-26,-21,-20,-22,-28,-37,-47,-57,-63,-63,-54,-44,-34,-26,-21,-20,-22,-28,-37,-47,-57,-63,-63,-54,-44,-34,-26,-21,-20,-22,-28,-37,-41.50,-41.5];
      | plot(A,B);
      | color('black');
      | port_label('LConn', 1, '+')
  848 Y Z : spsThreePhaseSeriesRLCLoadLib/Three-Phase Series RLC Load  LConnTagsString=A|B|C  Configuration=Y (grounded)  NominalVoltage=1000  Vabc=[ 1.0 1.0 1.0]*14376.02  Vabcp=[1e3 1e3 1e3]  NominalFrequency=60  UnbalancedPower=on  ActivePower=0  InductivePower=0  CapacitivePower=100  Pabc=[0 0 0]  QLabc=[0 0 0]  QCabc=[150 150 150]*1e3*a  Pabcp=[10e3 9e3 11e3]  QLabcp=[100 90 110]  QCabcp=[100 90 110]  Measurements=None  LoadType=constant Z
  850 : spsThreePhaseVIMeasurementLib/Three-Phase V-I Measurement  VoltageMeasurement=phase-to-ground  SetLabelV=on  LabelV=V850  Vpu=off  VpuLL=off  CurrentMeasurement=no  SetLabelI=off  LabelI=I815  Ipu=off  Pbase=100e6  Vbase=24900  OutputType=Complex  PhasorSimulation=on  PSBequivalent=0
  850-816 301 : spsThreePhasePISectionLineLib/Three-Phase PI Section Line  LConnTagsString=a|b|c  RConnTagsString=A|B|C  Length=310*ft2km  Frequency=60  Resistances=[R1_301 R0_301]  Inductances=[L1_301 L0_301]  Capacitances=[C1_301 C0_301]
  "852 " : spsThreePhaseVIMeasurementLib/Three-Phase V-I Measurement  VoltageMeasurement=phase-to-ground  SetLabelV=on  LabelV=V852  Vpu=off  VpuLL=off  CurrentMeasurement=no  SetLabelI=off  LabelI=I815  Ipu=off  Pbase=100e6  Vbase=24900  OutputType=Complex  PhasorSimulation=on  PSBequivalent=0
  852-832 301 : Subsystem  mask(Three-Phase PI Section Block){Rl=R_301, Ll=L_301, Cl=C_301, L=10*ft2km}
      mask prompts: Rl "Resistance per unit Length(Ohm/Km)[3x3 matrix]"; Ll "Inductance per unit Length(H/Km)[3x3 matrix]"; Cl "Capacitance per unit Length(F/Km)[3x3 matrix]"; L "Length (Km)"
      mask help: This block models a three-phase transmission line with a single PI section.
  854 : spsThreePhaseVIMeasurementLib/Three-Phase V-I Measurement  VoltageMeasurement=phase-to-ground  SetLabelV=on  LabelV=V854  Vpu=off  VpuLL=off  CurrentMeasurement=yes  SetLabelI=on  LabelI=I854  Ipu=off  Pbase=100e6  Vbase=24900  OutputType=Complex  PhasorSimulation=on  PSBequivalent=0
  854 Y PQ : Subsystem  mask(Single Phase ZIP Load){Vnom=1.0*14376.02, fnom=60, Pnom=4e3/2 *a, Qnom=2e3/2*a, LoadType=constant P, Vlim=0.7}
      mask prompts: Vnom "Nominal Voltage Vn (Vrms)"; fnom "Nominal Frequency fn (Hz)"; Pnom "Nominal Active power (W)"; Qnom "Nominal Reactive power (VAR)"; LoadType "Load Type"; Vlim "Minimum voltage (pu)"
      mask help:
      | Notes:
      | Single Phase ZIP load model which gets converted to constant Z type if the voltage becomes lower than the Minimum Voltage.
      mask TypeOptions LoadType: Constant Z | constant I | constant P
      mask DialogControl ParameterTabVar0 Prompt: Parameters
      mask DialogControl ParameterTabVar1 Prompt: Type
      mask Display:
      | color('red');
      | A=[-210,-180,-170,-160,-147,-140,-130,-120,-110,-80,-50,-49,-45,-39,-33,-26,-21,-18,-17,-19,-22,-22,-26,-27,-25,-22,-16,-9,-3,2,6,6,4,1,1,-3,-4,-2,2,7,14,20,26,29,30,28,24,24,21,20,21,25,31,37,44,49,50,50,80];
      | B=[-41.5,-41.5,-63,-20,-63,-20,-63,-20,-41.5,-41.5,-41.5,-34,-26,-21,-20,-22,-28,-37,-47,-57,-63,-63,-54,-44,-34,-26,-21,-20,-22,-28,-37,-47,-57,-63,-63,-54,-44,-34,-26,-21,-20,-22,-28,-37,-47,-57,-63,-63,-54,-44,-34,-26,-21,-20,-22,-28,-37,-41.50,-41.5];
      | plot(A,B);
      | color('black');
      | port_label('LConn', 1, '+')
  854-852 301 : Subsystem  mask(Three-Phase PI Section Block){Rl=R_301, Ll=L_301, Cl=C_301, L=36830*ft2km}
      mask prompts: Rl "Resistance per unit Length(Ohm/Km)[3x3 matrix]"; Ll "Inductance per unit Length(H/Km)[3x3 matrix]"; Cl "Capacitance per unit Length(F/Km)[3x3 matrix]"; L "Length (Km)"
      mask help: This block models a three-phase transmission line with a single PI section.
  854-856 303 : spsPiSectionLineLib/Pi Section Line  LConnTagsString=__new0  RConnTagsString=__new0  Phases=1  PiSections=1  Length=23330*ft2km  Frequency=60  Resistance=R1_303  Inductance=L1_303  Capacitance=C1_303  SpecifyConductance=off  Conductance=0  Measurements=None  Measurements2=None
      settings: LibrarySourceBlock=sps_lib/Power Grid Elements/Pi Section Line
  856 : Subsystem
  856 Y PQ : Subsystem  mask(Single Phase ZIP Load){Vnom=1.0*14376.02, fnom=60, Pnom=4e3/2 *a, Qnom=2e3/2*a, LoadType=constant P, Vlim=0.7}
      mask prompts: Vnom "Nominal Voltage Vn (Vrms)"; fnom "Nominal Frequency fn (Hz)"; Pnom "Nominal Active power (W)"; Qnom "Nominal Reactive power (VAR)"; LoadType "Load Type"; Vlim "Minimum voltage (pu)"
      mask help:
      | Notes:
      | Single Phase ZIP load model which gets converted to constant Z type if the voltage becomes lower than the Minimum Voltage.
      mask TypeOptions LoadType: Constant Z | constant I | constant P
      mask DialogControl ParameterTabVar0 Prompt: Parameters
      mask DialogControl ParameterTabVar1 Prompt: Type
      mask Display:
      | color('red');
      | A=[-210,-180,-170,-160,-147,-140,-130,-120,-110,-80,-50,-49,-45,-39,-33,-26,-21,-18,-17,-19,-22,-22,-26,-27,-25,-22,-16,-9,-3,2,6,6,4,1,1,-3,-4,-2,2,7,14,20,26,29,30,28,24,24,21,20,21,25,31,37,44,49,50,50,80];
      | B=[-41.5,-41.5,-63,-20,-63,-20,-63,-20,-41.5,-41.5,-41.5,-34,-26,-21,-20,-22,-28,-37,-47,-57,-63,-63,-54,-44,-34,-26,-21,-20,-22,-28,-37,-47,-57,-63,-63,-54,-44,-34,-26,-21,-20,-22,-28,-37,-47,-57,-63,-63,-54,-44,-34,-26,-21,-20,-22,-28,-37,-41.50,-41.5];
      | plot(A,B);
      | color('black');
      | port_label('LConn', 1, '+')
  858 : spsThreePhaseVIMeasurementLib/Three-Phase V-I Measurement  VoltageMeasurement=phase-to-ground  SetLabelV=on  LabelV=V858  Vpu=off  VpuLL=off  CurrentMeasurement=yes  SetLabelI=on  LabelI=I858  Ipu=off  Pbase=100e6  Vbase=24900  OutputType=Complex  PhasorSimulation=on  PSBequivalent=0
  858 D PQ : Subsystem  mask(Three Phase Delta ZIP Load (Phasor)){Vnom=24900, fnom=60, Pnom=[4 15 13]*1e3/2 *a, Qnom=[2 8 7]*1e3/2 *a, LoadType=Constant P, Vlim=0.7}
      mask prompts: Vnom "Nominal Ph-Ph Voltage (Vrms)"; fnom "Nominal Frequency fn (Hz)"; Pnom "Nominal Per Phase Active Power [Pab Pbc Pca] (W)"; Qnom "Nominal Per Phase Reactive Power [Qab Qbc Qca] (VAR)"; LoadType "Load Type"; Vlim "Minimum Voltage (pu)"
      mask help:
      | Notes:
      | Three Phase Delta Connected ZIP load model which gets converted to constant Z type if the voltage becomes lower than the Minimum Voltage.
      mask TypeOptions LoadType: Constant Z | Constant I | Constant P
      mask DialogControl ParameterTabVar0 Prompt: Parameters
      mask DialogControl ParameterTabVar01 Prompt: Type
      mask Display:
      | color('red');
      | %load figure 0deg
      | A=[-210,-180,-170,-160,-147,-140,-130,-120,-110,-80,-50,-49,-45,-39,-33,-26,-21,-18,-17,-19,-22,-22,-26,-27,-25,-22,-16,-9,-3,2,6,6,4,1,1,-3,-4,-2,2,7,14,20,26,29,30,28,24,24,21,20,21,25,31,37,44,49,50,50,80];
      | B=[-41.5,-41.5,-63,-20,-63,-20,-63,-20,-41.5,-41.5,-41.5,-34,-26,-21,-20,-22,-28,-37,-47,-57,-63,-63,-54,-44,-34,-26,-21,-20,-22,-28,-37,-47,-57,-63,-63,-54,-44,-34,-26,-21,-20,-22,-28,-37,-47,-57,-63,-63,-54,-44,-34,-26,-21,-20,-22,-28,-37,-41.50,-41.5];
      | plot(A,B);
      | 
      | %load figure 0deg inverted
      | A1=[-80,-50,-49,-45,-39,-33,-26,-21,-18,-17,-19,-22,-22,-26,-27,-25,-22,-16,-9,-3,2,6,6,4,1,1,-3,-4,-2,2,7,14,20,26,29,30,28,24,24,21,20,21,25,31,37,44,49,50,50,80,110,120,130,143,150,160,170,180,210];
      | B1=[-41.5,-41.5,-34,-26,-21,-20,-22,-28,-37,-47,-57,-63,-63,-54,-44,-34,-26,-21,-20,-22,-28,-37,-47,-57,-63,-63,-54,-44,-34,-26,-21,-20,-22,-28,-37,-47,-57,-63,-63,-54,-44,-34,-26,-21,-20,-22,-28,-37,-41.5,-41.5,-41.5,-63,-20,-63,-20,-63,-20,-41.5,-41.5];
      | 
      | 
      | %load figure -120deg
      | c=1*exp(sqrt(-1)*(-60*pi/180));
      | l=A1+j*B1;
      | m=l*c;
      | E=real(m);F=imag(m);
      | E=E+10.94;F=F+161.1;
      | plot(E,F);
      | 
      | %load figure +120deg
      | c=1*exp(sqrt(-1)*(60*pi/180));
      | l=A1+j*B1;
      | m=l*c;
      | G=real(m);
      | H=imag(m);
      | G=G-205.94;H=H+48.53;
      | plot(G,H);
      | 
      | color('black');
      | port_label('LConn', 1, 'A')
      | port_label('LConn', 2, 'B')
      | port_label('LConn', 3, 'C')
  858 D Z : Subsystem  mask(Three Phase Delta ZIP Load (Phasor)){Vnom=24900, fnom=60, Pnom=[7 2 6]*1e3/2 *a, Qnom=[3 1 3]*1e3/2*a, LoadType=Constant Z, Vlim=0.7}
      mask prompts: Vnom "Nominal Ph-Ph Voltage (Vrms)"; fnom "Nominal Frequency fn (Hz)"; Pnom "Nominal Per Phase Active Power [Pab Pbc Pca] (W)"; Qnom "Nominal Per Phase Reactive Power [Qab Qbc Qca] (VAR)"; LoadType "Load Type"; Vlim "Minimum Voltage (pu)"
      mask help:
      | Notes:
      | Three Phase Delta Connected ZIP load model which gets converted to constant Z type if the voltage becomes lower than the Minimum Voltage.
      mask TypeOptions LoadType: Constant Z | Constant I | Constant P
      mask DialogControl ParameterTabVar0 Prompt: Parameters
      mask DialogControl ParameterTabVar01 Prompt: Type
      mask Display:
      | color('red');
      | %load figure 0deg
      | A=[-210,-180,-170,-160,-147,-140,-130,-120,-110,-80,-50,-49,-45,-39,-33,-26,-21,-18,-17,-19,-22,-22,-26,-27,-25,-22,-16,-9,-3,2,6,6,4,1,1,-3,-4,-2,2,7,14,20,26,29,30,28,24,24,21,20,21,25,31,37,44,49,50,50,80];
      | B=[-41.5,-41.5,-63,-20,-63,-20,-63,-20,-41.5,-41.5,-41.5,-34,-26,-21,-20,-22,-28,-37,-47,-57,-63,-63,-54,-44,-34,-26,-21,-20,-22,-28,-37,-47,-57,-63,-63,-54,-44,-34,-26,-21,-20,-22,-28,-37,-47,-57,-63,-63,-54,-44,-34,-26,-21,-20,-22,-28,-37,-41.50,-41.5];
      | plot(A,B);
      | 
      | %load figure 0deg inverted
      | A1=[-80,-50,-49,-45,-39,-33,-26,-21,-18,-17,-19,-22,-22,-26,-27,-25,-22,-16,-9,-3,2,6,6,4,1,1,-3,-4,-2,2,7,14,20,26,29,30,28,24,24,21,20,21,25,31,37,44,49,50,50,80,110,120,130,143,150,160,170,180,210];
      | B1=[-41.5,-41.5,-34,-26,-21,-20,-22,-28,-37,-47,-57,-63,-63,-54,-44,-34,-26,-21,-20,-22,-28,-37,-47,-57,-63,-63,-54,-44,-34,-26,-21,-20,-22,-28,-37,-47,-57,-63,-63,-54,-44,-34,-26,-21,-20,-22,-28,-37,-41.5,-41.5,-41.5,-63,-20,-63,-20,-63,-20,-41.5,-41.5];
      | 
      | 
      | %load figure -120deg
      | c=1*exp(sqrt(-1)*(-60*pi/180));
      | l=A1+j*B1;
      | m=l*c;
      | E=real(m);F=imag(m);
      | E=E+10.94;F=F+161.1;
      | plot(E,F);
      | 
      | %load figure +120deg
      | c=1*exp(sqrt(-1)*(60*pi/180));
      | l=A1+j*B1;
      | m=l*c;
      | G=real(m);
      | H=imag(m);
      | G=G-205.94;H=H+48.53;
      | plot(G,H);
      | 
      | color('black');
      | port_label('LConn', 1, 'A')
      | port_label('LConn', 2, 'B')
      | port_label('LConn', 3, 'C')
  858 Y PQ : Subsystem  mask(Single Phase ZIP Load){Vnom=1.0*14376.02, fnom=60, Pnom=2e3/2*a, Qnom=1e3/2*a, LoadType=constant P, Vlim=0.7}
      mask prompts: Vnom "Nominal Voltage Vn (Vrms)"; fnom "Nominal Frequency fn (Hz)"; Pnom "Nominal Active power (W)"; Qnom "Nominal Reactive power (VAR)"; LoadType "Load Type"; Vlim "Minimum voltage (pu)"
      mask help:
      | Notes:
      | Single Phase ZIP load model which gets converted to constant Z type if the voltage becomes lower than the Minimum Voltage.
      mask TypeOptions LoadType: Constant Z | constant I | constant P
      mask DialogControl ParameterTabVar0 Prompt: Parameters
      mask DialogControl ParameterTabVar1 Prompt: Type
      mask Display:
      | color('red');
      | A=[-210,-180,-170,-160,-147,-140,-130,-120,-110,-80,-50,-49,-45,-39,-33,-26,-21,-18,-17,-19,-22,-22,-26,-27,-25,-22,-16,-9,-3,2,6,6,4,1,1,-3,-4,-2,2,7,14,20,26,29,30,28,24,24,21,20,21,25,31,37,44,49,50,50,80];
      | B=[-41.5,-41.5,-63,-20,-63,-20,-63,-20,-41.5,-41.5,-41.5,-34,-26,-21,-20,-22,-28,-37,-47,-57,-63,-63,-54,-44,-34,-26,-21,-20,-22,-28,-37,-47,-57,-63,-63,-54,-44,-34,-26,-21,-20,-22,-28,-37,-47,-57,-63,-63,-54,-44,-34,-26,-21,-20,-22,-28,-37,-41.50,-41.5];
      | plot(A,B);
      | color('black');
      | port_label('LConn', 1, '+')
  858-834 301 : spsThreePhasePISectionLineLib/Three-Phase PI Section Line  LConnTagsString=a|b|c  RConnTagsString=A|B|C  Length=5830*ft2km  Frequency=60  Resistances=[R1_301 R0_301]  Inductances=[L1_301 L0_301]  Capacitances=[C1_301 C0_301]
  858-864 302 : spsPiSectionLineLib/Pi Section Line  LConnTagsString=__new0  RConnTagsString=__new0  Phases=1  PiSections=1  Length=1620*ft2km  Frequency=60  Resistance=R1_302  Inductance=L1_302  Capacitance=C1_302  SpecifyConductance=off  Conductance=0  Measurements=None  Measurements2=None
      settings: LibrarySourceBlock=sps_lib/Power Grid Elements/Pi Section Line
  860 : spsThreePhaseVIMeasurementLib/Three-Phase V-I Measurement  VoltageMeasurement=phase-to-ground  SetLabelV=on  LabelV=V860  Vpu=off  VpuLL=off  CurrentMeasurement=no  SetLabelI=on  LabelI=I860  Ipu=off  Pbase=100e6  Vbase=24900  OutputType=Complex  PhasorSimulation=on  PSBequivalent=0
  860 D PQ : Subsystem  mask(Three Phase Delta ZIP Load (Phasor)){Vnom=24900, fnom=60, Pnom=[30 10 42]*1e3/2 *a, Qnom=[15 6 22]*1e3/2 *a, LoadType=Constant P, Vlim=0.7}
      mask prompts: Vnom "Nominal Ph-Ph Voltage (Vrms)"; fnom "Nominal Frequency fn (Hz)"; Pnom "Nominal Per Phase Active Power [Pab Pbc Pca] (W)"; Qnom "Nominal Per Phase Reactive Power [Qab Qbc Qca] (VAR)"; LoadType "Load Type"; Vlim "Minimum Voltage (pu)"
      mask help:
      | Notes:
      | Three Phase Delta Connected ZIP load model which gets converted to constant Z type if the voltage becomes lower than the Minimum Voltage.
      mask TypeOptions LoadType: Constant Z | Constant I | Constant P
      mask DialogControl ParameterTabVar0 Prompt: Parameters
      mask DialogControl ParameterTabVar01 Prompt: Type
      mask Display:
      | color('red');
      | %load figure 0deg
      | A=[-210,-180,-170,-160,-147,-140,-130,-120,-110,-80,-50,-49,-45,-39,-33,-26,-21,-18,-17,-19,-22,-22,-26,-27,-25,-22,-16,-9,-3,2,6,6,4,1,1,-3,-4,-2,2,7,14,20,26,29,30,28,24,24,21,20,21,25,31,37,44,49,50,50,80];
      | B=[-41.5,-41.5,-63,-20,-63,-20,-63,-20,-41.5,-41.5,-41.5,-34,-26,-21,-20,-22,-28,-37,-47,-57,-63,-63,-54,-44,-34,-26,-21,-20,-22,-28,-37,-47,-57,-63,-63,-54,-44,-34,-26,-21,-20,-22,-28,-37,-47,-57,-63,-63,-54,-44,-34,-26,-21,-20,-22,-28,-37,-41.50,-41.5];
      | plot(A,B);
      | 
      | %load figure 0deg inverted
      | A1=[-80,-50,-49,-45,-39,-33,-26,-21,-18,-17,-19,-22,-22,-26,-27,-25,-22,-16,-9,-3,2,6,6,4,1,1,-3,-4,-2,2,7,14,20,26,29,30,28,24,24,21,20,21,25,31,37,44,49,50,50,80,110,120,130,143,150,160,170,180,210];
      | B1=[-41.5,-41.5,-34,-26,-21,-20,-22,-28,-37,-47,-57,-63,-63,-54,-44,-34,-26,-21,-20,-22,-28,-37,-47,-57,-63,-63,-54,-44,-34,-26,-21,-20,-22,-28,-37,-47,-57,-63,-63,-54,-44,-34,-26,-21,-20,-22,-28,-37,-41.5,-41.5,-41.5,-63,-20,-63,-20,-63,-20,-41.5,-41.5];
      | 
      | 
      | %load figure -120deg
      | c=1*exp(sqrt(-1)*(-60*pi/180));
      | l=A1+j*B1;
      | m=l*c;
      | E=real(m);F=imag(m);
      | E=E+10.94;F=F+161.1;
      | plot(E,F);
      | 
      | %load figure +120deg
      | c=1*exp(sqrt(-1)*(60*pi/180));
      | l=A1+j*B1;
      | m=l*c;
      | G=real(m);
      | H=imag(m);
      | G=G-205.94;H=H+48.53;
      | plot(G,H);
      | 
      | color('black');
      | port_label('LConn', 1, 'A')
      | port_label('LConn', 2, 'B')
      | port_label('LConn', 3, 'C')
  860 D Z : Subsystem  mask(Three Phase Delta ZIP Load (Phasor)){Vnom=24900, fnom=60, Pnom=[16 20 110]*1e3/2 *a, Qnom=[8 10 55]*1e3/2*a, LoadType=Constant Z, Vlim=0.7}
      mask prompts: Vnom "Nominal Ph-Ph Voltage (Vrms)"; fnom "Nominal Frequency fn (Hz)"; Pnom "Nominal Per Phase Active Power [Pab Pbc Pca] (W)"; Qnom "Nominal Per Phase Reactive Power [Qab Qbc Qca] (VAR)"; LoadType "Load Type"; Vlim "Minimum Voltage (pu)"
      mask help:
      | Notes:
      | Three Phase Delta Connected ZIP load model which gets converted to constant Z type if the voltage becomes lower than the Minimum Voltage.
      mask TypeOptions LoadType: Constant Z | Constant I | Constant P
      mask DialogControl ParameterTabVar0 Prompt: Parameters
      mask DialogControl ParameterTabVar01 Prompt: Type
      mask Display:
      | color('red');
      | %load figure 0deg
      | A=[-210,-180,-170,-160,-147,-140,-130,-120,-110,-80,-50,-49,-45,-39,-33,-26,-21,-18,-17,-19,-22,-22,-26,-27,-25,-22,-16,-9,-3,2,6,6,4,1,1,-3,-4,-2,2,7,14,20,26,29,30,28,24,24,21,20,21,25,31,37,44,49,50,50,80];
      | B=[-41.5,-41.5,-63,-20,-63,-20,-63,-20,-41.5,-41.5,-41.5,-34,-26,-21,-20,-22,-28,-37,-47,-57,-63,-63,-54,-44,-34,-26,-21,-20,-22,-28,-37,-47,-57,-63,-63,-54,-44,-34,-26,-21,-20,-22,-28,-37,-47,-57,-63,-63,-54,-44,-34,-26,-21,-20,-22,-28,-37,-41.50,-41.5];
      | plot(A,B);
      | 
      | %load figure 0deg inverted
      | A1=[-80,-50,-49,-45,-39,-33,-26,-21,-18,-17,-19,-22,-22,-26,-27,-25,-22,-16,-9,-3,2,6,6,4,1,1,-3,-4,-2,2,7,14,20,26,29,30,28,24,24,21,20,21,25,31,37,44,49,50,50,80,110,120,130,143,150,160,170,180,210];
      | B1=[-41.5,-41.5,-34,-26,-21,-20,-22,-28,-37,-47,-57,-63,-63,-54,-44,-34,-26,-21,-20,-22,-28,-37,-47,-57,-63,-63,-54,-44,-34,-26,-21,-20,-22,-28,-37,-47,-57,-63,-63,-54,-44,-34,-26,-21,-20,-22,-28,-37,-41.5,-41.5,-41.5,-63,-20,-63,-20,-63,-20,-41.5,-41.5];
      | 
      | 
      | %load figure -120deg
      | c=1*exp(sqrt(-1)*(-60*pi/180));
      | l=A1+j*B1;
      | m=l*c;
      | E=real(m);F=imag(m);
      | E=E+10.94;F=F+161.1;
      | plot(E,F);
      | 
      | %load figure +120deg
      | c=1*exp(sqrt(-1)*(60*pi/180));
      | l=A1+j*B1;
      | m=l*c;
      | G=real(m);
      | H=imag(m);
      | G=G-205.94;H=H+48.53;
      | plot(G,H);
      | 
      | color('black');
      | port_label('LConn', 1, 'A')
      | port_label('LConn', 2, 'B')
      | port_label('LConn', 3, 'C')
  860 Y PQ : Subsystem  mask(Three Phase Star ZIP Load (Phasor)){Vnom=24900, fnom=60, Pnom=[20 20 20]*1e3 *a, Qnom=[16 16 16]*1e3*a, LoadType=Constant P, Vlim=0.7}
      mask prompts: Vnom "Nominal Ph-Ph voltage (Vrms)"; fnom "Nominal Frequency fn (Hz)"; Pnom "Nominal Per Phase Active Power [Pa Pb Pc] (W)"; Qnom "Nominal Per Phase Reactive Power [Qa Qb Qc] (VAR)"; LoadType "Load Type"; Vlim "Minimum voltage (pu)"
      mask help:
      | Notes:
      | Three Phase Star Connected ZIP load model which gets converted to constant Z type if the voltage becomes lower than the Minimum Voltage.
      mask TypeOptions LoadType: Constant Z | Constant I | Constant P
      mask DialogControl ParameterTabVar0 Prompt: Parameters
      mask DialogControl ParameterTabVar01 Prompt: Type
      mask Display:
      | color('red');
      | %load figure 0deg
      | A=[-210,-180,-170,-160,-147,-140,-130,-120,-110,-80,-50,-49,-45,-39,-33,-26,-21,-18,-17,-19,-22,-22,-26,-27,-25,-22,-16,-9,-3,2,6,6,4,1,1,-3,-4,-2,2,7,14,20,26,29,30,28,24,24,21,20,21,25,31,37,44,49,50,50,80];
      | B=[-41.5,-41.5,-63,-20,-63,-20,-63,-20,-41.5,-41.5,-41.5,-34,-26,-21,-20,-22,-28,-37,-47,-57,-63,-63,-54,-44,-34,-26,-21,-20,-22,-28,-37,-47,-57,-63,-63,-54,-44,-34,-26,-21,-20,-22,-28,-37,-47,-57,-63,-63,-54,-44,-34,-26,-21,-20,-22,-28,-37,-41.50,-41.5];
      | % plot(A,B);
      | 
      | %load figure 0deg inverted
      | A1=[-80,-50,-49,-45,-39,-33,-26,-21,-18,-17,-19,-22,-22,-26,-27,-25,-22,-16,-9,-3,2,6,6,4,1,1,-3,-4,-2,2,7,14,20,26,29,30,28,24,24,21,20,21,25,31,37,44,49,50,50,80,110,120,130,143,150,160,170,180,210];
      | B1=[-41.5,-41.5,-34,-26,-21,-20,-22,-28,-37,-47,-57,-63,-63,-54,-44,-34,-26,-21,-20,-22,-28,-37,-47,-57,-63,-63,-54,-44,-34,-26,-21,-20,-22,-28,-37,-47,-57,-63,-63,-54,-44,-34,-26,-21,-20,-22,-28,-37,-41.5,-41.5,-41.5,-63,-20,-63,-20,-63,-20,-41.5,-41.5];
      | 
      | 
      | %load figure 90deg
      | C=[-41.5,-41.5,-20,-63,-20,-63,-20,-63,-41.5,-41.5,-41.5,-37,-28,-22,-20,-21,-26,-34,-44,-54,-63,-63,-57,-47,-37,-28,-22,-20,-21,-26,-34,-44,-54,-63,-63,-57,-47,-37,-28,-22,-20,-21,-26,-34,-44,-54,-63,-63,-57,-47,-37,-28,-22,-20,-21,-26,-34,-41.5,-41.5];
      | D=[190,160,150,140,130,123,110,100,90,80,50,50,49,44,37,31,25,21,20,21,24,24,28,30,29,26,20,14,7,2,-2,-4,-3,1,1,4,6,6,2,-3,-9,-16,-22,-25,-27,-26,-22,-22,-19,-17,-18,-21,-26,-33,-39,-45,-49,-50,-70];
      | plot(C,D);
      | 
      | 
      | %load figure -120deg
      | c=1*exp(sqrt(-1)*(-60*pi/180));
      | l=A1+j*B1;
      | m=l*c;
      | E=real(m);F=imag(m);
      | E=E+34.4400;F=F-118.53;
      | plot(E,F);
      | 
      | %load figure +120deg
      | c=1*exp(sqrt(-1)*(60*pi/180));
      | l=A+j*B;
      | m=l*c;
      | G=real(m);
      | H=imag(m);
      | G=G-117.44;H=H-118.5300;
      | plot(G,H);
      | 
      | color('black');
      | port_label('LConn', 1, 'A')
      | port_label('LConn', 2, 'B')
      | port_label('LConn', 3, 'C')
  860-836 301 : spsThreePhasePISectionLineLib/Three-Phase PI Section Line  LConnTagsString=a|b|c  RConnTagsString=A|B|C  Length=2680*ft2km  Frequency=60  Resistances=[R1_301 R0_301]  Inductances=[L1_301 L0_301]  Capacitances=[C1_301 C0_301]
  862 : spsThreePhaseVIMeasurementLib/Three-Phase V-I Measurement  VoltageMeasurement=phase-to-ground  SetLabelV=on  LabelV=V862  Vpu=off  VpuLL=off  CurrentMeasurement=yes  SetLabelI=on  LabelI=I862  Ipu=off  Pbase=100e6  Vbase=24900  OutputType=Complex  PhasorSimulation=on  PSBequivalent=0
  862 Y PQ : Subsystem  mask(Single Phase ZIP Load){Vnom=1.0*14376.02, fnom=60, Pnom=28e3/2 *a, Qnom=14e3/2*a, LoadType=constant P, Vlim=0.7}
      mask prompts: Vnom "Nominal Voltage Vn (Vrms)"; fnom "Nominal Frequency fn (Hz)"; Pnom "Nominal Active power (W)"; Qnom "Nominal Reactive power (VAR)"; LoadType "Load Type"; Vlim "Minimum voltage (pu)"
      mask help:
      | Notes:
      | Single Phase ZIP load model which gets converted to constant Z type if the voltage becomes lower than the Minimum Voltage.
      mask TypeOptions LoadType: Constant Z | constant I | constant P
      mask DialogControl ParameterTabVar0 Prompt: Parameters
      mask DialogControl ParameterTabVar1 Prompt: Type
      mask Display:
      | color('red');
      | A=[-210,-180,-170,-160,-147,-140,-130,-120,-110,-80,-50,-49,-45,-39,-33,-26,-21,-18,-17,-19,-22,-22,-26,-27,-25,-22,-16,-9,-3,2,6,6,4,1,1,-3,-4,-2,2,7,14,20,26,29,30,28,24,24,21,20,21,25,31,37,44,49,50,50,80];
      | B=[-41.5,-41.5,-63,-20,-63,-20,-63,-20,-41.5,-41.5,-41.5,-34,-26,-21,-20,-22,-28,-37,-47,-57,-63,-63,-54,-44,-34,-26,-21,-20,-22,-28,-37,-47,-57,-63,-63,-54,-44,-34,-26,-21,-20,-22,-28,-37,-47,-57,-63,-63,-54,-44,-34,-26,-21,-20,-22,-28,-37,-41.50,-41.5];
      | plot(A,B);
      | color('black');
      | port_label('LConn', 1, '+')
  862-838 304 : spsPiSectionLineLib/Pi Section Line  LConnTagsString=__new0  RConnTagsString=__new0  Phases=1  PiSections=1  Length=4860*ft2km  Frequency=60  Resistance=R1_304  Inductance=L1_304  Capacitance=C1_304  SpecifyConductance=off  Conductance=0  Measurements=None  Measurements2=None
      settings: LibrarySourceBlock=sps_lib/Power Grid Elements/Pi Section Line
  864 : Subsystem
  864 Y PQ : Subsystem  mask(Single Phase ZIP Load){Vnom=1.0*14376.02, fnom=60, Pnom=2e3/2 *a, Qnom=1e3/2*a, LoadType=constant P, Vlim=0.7}
      mask prompts: Vnom "Nominal Voltage Vn (Vrms)"; fnom "Nominal Frequency fn (Hz)"; Pnom "Nominal Active power (W)"; Qnom "Nominal Reactive power (VAR)"; LoadType "Load Type"; Vlim "Minimum voltage (pu)"
      mask help:
      | Notes:
      | Single Phase ZIP load model which gets converted to constant Z type if the voltage becomes lower than the Minimum Voltage.
      mask TypeOptions LoadType: Constant Z | constant I | constant P
      mask DialogControl ParameterTabVar0 Prompt: Parameters
      mask DialogControl ParameterTabVar1 Prompt: Type
      mask Display:
      | color('red');
      | A=[-210,-180,-170,-160,-147,-140,-130,-120,-110,-80,-50,-49,-45,-39,-33,-26,-21,-18,-17,-19,-22,-22,-26,-27,-25,-22,-16,-9,-3,2,6,6,4,1,1,-3,-4,-2,2,7,14,20,26,29,30,28,24,24,21,20,21,25,31,37,44,49,50,50,80];
      | B=[-41.5,-41.5,-63,-20,-63,-20,-63,-20,-41.5,-41.5,-41.5,-34,-26,-21,-20,-22,-28,-37,-47,-57,-63,-63,-54,-44,-34,-26,-21,-20,-22,-28,-37,-47,-57,-63,-63,-54,-44,-34,-26,-21,-20,-22,-28,-37,-47,-57,-63,-63,-54,-44,-34,-26,-21,-20,-22,-28,-37,-41.50,-41.5];
      | plot(A,B);
      | color('black');
      | port_label('LConn', 1, '+')
  888 : spsThreePhaseVIMeasurementLib/Three-Phase V-I Measurement  VoltageMeasurement=phase-to-ground  SetLabelV=on  LabelV=V888  Vpu=off  VpuLL=off  CurrentMeasurement=yes  SetLabelI=on  LabelI=I888  Ipu=off  Pbase=100e6  Vbase=24900  OutputType=Complex  PhasorSimulation=on  PSBequivalent=0
  888-890 300 : spsThreePhasePISectionLineLib/Three-Phase PI Section Line  LConnTagsString=a|b|c  RConnTagsString=A|B|C  Length=10560*ft2km  Frequency=60  Resistances=[R1_300 R0_300]  Inductances=[L1_300 L0_300]  Capacitances=[C1_300 C0_300]
  890 : spsThreePhaseVIMeasurementLib/Three-Phase V-I Measurement  VoltageMeasurement=phase-to-ground  SetLabelV=on  LabelV=V890  Vpu=off  VpuLL=off  CurrentMeasurement=yes  SetLabelI=on  LabelI=I890  Ipu=off  Pbase=100e6  Vbase=4160  OutputType=Complex  PhasorSimulation=on  PSBequivalent=0
  890 D I : Subsystem  mask(Three Phase Delta ZIP Load (Phasor)){Vnom=4160, fnom=60, Pnom=[150 150 150]*1e3 *a, Qnom=[75 75 75]*1e3 *a, LoadType=Constant I, Vlim=0.7}
      mask prompts: Vnom "Nominal Ph-Ph Voltage (Vrms)"; fnom "Nominal Frequency fn (Hz)"; Pnom "Nominal Per Phase Active Power [Pab Pbc Pca] (W)"; Qnom "Nominal Per Phase Reactive Power [Qab Qbc Qca] (VAR)"; LoadType "Load Type"; Vlim "Minimum Voltage (pu)"
      mask help:
      | Notes:
      | Three Phase Delta Connected ZIP load model which gets converted to constant Z type if the voltage becomes lower than the Minimum Voltage.
      mask TypeOptions LoadType: Constant Z | Constant I | Constant P
      mask DialogControl ParameterTabVar0 Prompt: Parameters
      mask DialogControl ParameterTabVar01 Prompt: Type
      mask Display:
      | color('red');
      | %load figure 0deg
      | A=[-210,-180,-170,-160,-147,-140,-130,-120,-110,-80,-50,-49,-45,-39,-33,-26,-21,-18,-17,-19,-22,-22,-26,-27,-25,-22,-16,-9,-3,2,6,6,4,1,1,-3,-4,-2,2,7,14,20,26,29,30,28,24,24,21,20,21,25,31,37,44,49,50,50,80];
      | B=[-41.5,-41.5,-63,-20,-63,-20,-63,-20,-41.5,-41.5,-41.5,-34,-26,-21,-20,-22,-28,-37,-47,-57,-63,-63,-54,-44,-34,-26,-21,-20,-22,-28,-37,-47,-57,-63,-63,-54,-44,-34,-26,-21,-20,-22,-28,-37,-47,-57,-63,-63,-54,-44,-34,-26,-21,-20,-22,-28,-37,-41.50,-41.5];
      | plot(A,B);
      | 
      | %load figure 0deg inverted
      | A1=[-80,-50,-49,-45,-39,-33,-26,-21,-18,-17,-19,-22,-22,-26,-27,-25,-22,-16,-9,-3,2,6,6,4,1,1,-3,-4,-2,2,7,14,20,26,29,30,28,24,24,21,20,21,25,31,37,44,49,50,50,80,110,120,130,143,150,160,170,180,210];
      | B1=[-41.5,-41.5,-34,-26,-21,-20,-22,-28,-37,-47,-57,-63,-63,-54,-44,-34,-26,-21,-20,-22,-28,-37,-47,-57,-63,-63,-54,-44,-34,-26,-21,-20,-22,-28,-37,-47,-57,-63,-63,-54,-44,-34,-26,-21,-20,-22,-28,-37,-41.5,-41.5,-41.5,-63,-20,-63,-20,-63,-20,-41.5,-41.5];
      | 
      | 
      | %load figure -120deg
      | c=1*exp(sqrt(-1)*(-60*pi/180));
      | l=A1+j*B1;
      | m=l*c;
      | E=real(m);F=imag(m);
      | E=E+10.94;F=F+161.1;
      | plot(E,F);
      | 
      | %load figure +120deg
      | c=1*exp(sqrt(-1)*(60*pi/180));
      | l=A1+j*B1;
      | m=l*c;
      | G=real(m);
      | H=imag(m);
      | G=G-205.94;H=H+48.53;
      | plot(G,H);
      | 
      | color('black');
      | port_label('LConn', 1, 'A')
      | port_label('LConn', 2, 'B')
      | port_label('LConn', 3, 'C')
  Ground{1..22} (22 alike) : spsGroundLib/Ground  LConnTagsString=a
  Node Voltages : Subsystem
  RG10 : spsThreePhaseVIMeasurementLib/Three-Phase V-I Measurement  VoltageMeasurement=phase-to-ground  SetLabelV=on  LabelV=RG10  Vpu=off  VpuLL=off  CurrentMeasurement=no  SetLabelI=off  LabelI=I815  Ipu=off  Pbase=100e6  Vbase=24900  OutputType=Complex  PhasorSimulation=on  PSBequivalent=0
  RG11 : spsThreePhaseVIMeasurementLib/Three-Phase V-I Measurement  VoltageMeasurement=phase-to-ground  SetLabelV=on  LabelV=RG11  Vpu=off  VpuLL=off  CurrentMeasurement=no  SetLabelI=off  LabelI=I815  Ipu=off  Pbase=100e6  Vbase=24900  OutputType=Complex  PhasorSimulation=on  PSBequivalent=0
  Regulator 1 : Subsystem
  Regulator 2 : Subsystem
  Regulator Taps : Subsystem
  Series RLC Branch3 : spsSeriesRLCBranchLib/Series RLC Branch  LConnTagsString=__new0  RConnTagsString=__new0  BranchType=R  Resistance=.001  Inductance=0  SetiL0=off  InitialCurrent=0  Capacitance=0  Setx0=off  InitialVoltage=0  Measurements=None
  Series RLC Branch4 : spsSeriesRLCBranchLib/Series RLC Branch  LConnTagsString=__new0  RConnTagsString=__new0  BranchType=R  Resistance=.001  Inductance=0  SetiL0=off  InitialCurrent=0  Capacitance=0  Setx0=off  InitialVoltage=0  Measurements=None
  Series RLC Branch5 : spsSeriesRLCBranchLib/Series RLC Branch  LConnTagsString=__new0  RConnTagsString=__new0  BranchType=R  Resistance=.001  Inductance=0  SetiL0=off  InitialCurrent=0  Capacitance=0  Setx0=off  InitialVoltage=0  Measurements=None
  Substation Power : Subsystem
  Three-Phase Transformer (Two Windings)1 : spsThreePhaseTransformerTwoWindingsLib/Three-Phase Transformer (Two Windings)  Winding1Connection=Yg  Winding2Connection=Yg  CoreType=Three single-phase transformers  SetSaturation=off  Hysteresis=off  DataFile='hysteresis'  SetInitialFlux=on  Measurements=None  UNITS=pu  NominalPower=[ 500e3 , 60 ]  Winding1=[24900 0.019 0.0408]  Winding2=[4160 1e-4 1e-3]  Rm=500  Lm=500  L0=0.5  Saturation="[0 0; 0.0 1.2; 1.0  1.52]"  InitialFluxes="[0.8  -0.4  0.4]"  BreakLoop=off  DiscreteSolver=Trapezoidal iterative  DataType=off  TransfoNumber=1
  Three-Phase Source : spsThreePhaseSourceLib/Three-Phase Source  InternalConnection=Yg  VoltagePhases=on  Voltage=25e3  PhaseAngle=0  Voltage_phases=[ 1.05 1.05 1.05]*14376.02  PhaseAngles_phases=[ 0 -120 120]  Frequency=60  NonIdealSource=off  SpecifyImpedance=off  Resistance=1e-6  Inductance=1e-5  ShortCircuitLevel=100e6  BaseVoltage=24.9e3  XRratio=7  BusType=swing  Pref=10e3  Qref=0  Prefabc=[10e3, 10e3, 10e3]  Qrefabc=[0, 0, 0]  Qmin=-inf  Qmax=inf
  XF10 : spsThreePhaseVIMeasurementLib/Three-Phase V-I Measurement  VoltageMeasurement=phase-to-ground  SetLabelV=on  LabelV=XF10  Vpu=off  VpuLL=off  CurrentMeasurement=no  SetLabelI=on  LabelI=I888  Ipu=off  Pbase=100e6  Vbase=24900  OutputType=Complex  PhasorSimulation=on  PSBequivalent=0
  powergui : spspowerguiLib/powergui  Priority=1  SimulationMode=Phasor  SampleTime=Ts  frequency=60  Iterations=50  frequencyindice=60  Pbase=100e6  ErrMax=1e-4  UnitsV=kV  UnitsW=MW  buscounter=0  FunctionMessages=off  echomessages=on  EnableUseOfTLC=off  CurrentSourceSwitches=off  DisableSnubberDevices=off  DisableRonSwitches=off  DisableVfSwitches=off  DisplayEquations=off  AutomaticDiscreteSolvers=off  SolverType=Tustin  Interpol=off  ExternalGateDelay=off  methode=off  Ts=0  x0status=blocks  SPID=off  SwTol=0  HookPort=off  NonlinearTolerance=1e-4  nMaxIteration=100  ContinueOnMaxIteration=off  RestoreLinks=warning  ResistiveCurrentMeasurement=off  Frange=[0:2:500]  Ylog=off  Xlog=on  ShowGrid=off  save=off  variable=ZData  structure=0  ZoomFFT=off  StartTime=0.0  cycles=1  DisplayStyle=1  fundamental=60  FreqAxis=off  MaxFrequency=1000  frequencyindicesteady=1  RmsSteady=1  display=off
  tag scope: Reg1=global, Reg2=global
  wires:
  Regulator 2/1(Tap) -> [Reg2]
  Regulator 1/1(Tap) -> [Reg1]
  connections:
  838 Y PQ/LConn1 -- 838/LConn1
  838/RConn1 -- 862-838 304/RConn1
  856 Y PQ/LConn1 -- 856/LConn1
  856/RConn1 -- 854-856 303/RConn1
  864 Y PQ/LConn1 -- 864/LConn1
  864/RConn1 -- 858-864 302/RConn1
  826 Y I/LConn1 -- 826/LConn1
  826/RConn1 -- 824-826 303/RConn1
  822 Y PQ/LConn1 -- 822/LConn1
  822/RConn1 -- 820-822 302/RConn1
  818-820 302/RConn1 -- 820Y Z/LConn1 -- 820/RConn1
  818/RConn1 -- 816-818 302/RConn1
  810 Y I/LConn1 -- 810/LConn1
  810/RConn1 -- 808-810 303/RConn1
  Regulator 2/RConn1 -- RG11/LConn1
  Regulator 2/RConn2 -- RG11/LConn2
  Regulator 2/RConn3 -- RG11/LConn3
  Regulator 2/LConn3 -- "852 "/RConn3
  Regulator 2/LConn2 -- "852 "/RConn2
  Regulator 2/LConn1 -- "852 "/RConn1
  832-858 301/LConn1 -- 832/RConn1 -- Three-Phase Transformer (Two Windings)1/LConn1 -- 832 D Z/LConn1
  832-858 301/LConn2 -- Three-Phase Transformer (Two Windings)1/LConn2 -- 832/RConn2 -- 832 D Z/LConn2
  832-858 301/LConn3 -- Three-Phase Transformer (Two Windings)1/LConn3 -- 832/RConn3 -- 832 D Z/LConn3
  XF10/RConn3 -- 888/LConn3
  XF10/RConn2 -- 888/LConn2
  XF10/RConn1 -- 888/LConn1
  852-832 301/RConn3 -- 832/LConn3
  852-832 301/RConn2 -- 832/LConn2
  852-832 301/RConn1 -- 832/LConn1
  814-850 301/RConn3 -- 850/LConn3
  814-850 301/RConn2 -- 850/LConn2
  814-850 301/RConn1 -- 850/LConn1
  814-850 301/LConn3 -- RG10/RConn3
  814-850 301/LConn2 -- RG10/RConn2
  814-850 301/LConn1 -- RG10/RConn1
  Regulator 1/RConn1 -- RG10/LConn1
  812-814 300/RConn2 -- 814/LConn2
  812-814 300/RConn1 -- 814/LConn1
  812-814 300/RConn3 -- 814/LConn3
  852-832 301/LConn3 -- RG11/RConn3
  852-832 301/LConn2 -- RG11/RConn2
  852-832 301/LConn1 -- RG11/RConn1
  Regulator 1/RConn2 -- RG10/LConn2
  850/RConn1 -- 850-816 301/LConn1
  Regulator 1/RConn3 -- RG10/LConn3
  Regulator 1/LConn2 -- 814/RConn2
  Regulator 1/LConn3 -- 814/RConn3
  Regulator 1/LConn1 -- 814/RConn1
  850/RConn2 -- 850-816 301/LConn2
  850/RConn3 -- 850-816 301/LConn3
  812-814 300/LConn3 -- 812/RConn3
  812-814 300/LConn2 -- 812/RConn2
  812-814 300/LConn1 -- 812/RConn1
  812/LConn3 -- 808-812 300/RConn3
  812/LConn2 -- 808-812 300/RConn2
  812/LConn1 -- 808-812 300/RConn1
  858 D Z/LConn2 -- 858/RConn2 -- 858 D PQ/LConn2 -- 858-834 301/LConn2
  858 D Z/LConn1 -- 858/RConn1 -- 858 Y PQ/LConn1 -- 858 D PQ/LConn1 -- 858-834 301/LConn1 -- 858-864 302/LConn1
  800/RConn3 -- Series RLC Branch5/LConn1
  Series RLC Branch3/RConn1 -- 800-802 300/LConn1
  800/RConn2 -- Series RLC Branch4/LConn1
  Series RLC Branch5/RConn1 -- 800-802 300/LConn3
  Series RLC Branch4/RConn1 -- 800-802 300/LConn2
  800/RConn1 -- Series RLC Branch3/LConn1
  890 D I/LConn1 -- 890/RConn1
  890 D I/LConn3 -- 890/RConn3
  890 D I/LConn2 -- 890/RConn2
  890/LConn2 -- 888-890 300/RConn2
  888/RConn3 -- 888-890 300/LConn3
  890/LConn1 -- 888-890 300/RConn1
  800/LConn2 -- Three-Phase Source/RConn2
  800/LConn3 -- Three-Phase Source/RConn3
  800/LConn1 -- Three-Phase Source/RConn1
  890/LConn3 -- 888-890 300/RConn3
  888/RConn2 -- 888-890 300/LConn2
  842/LConn2 -- 834-842 301/RConn2
  842/LConn1 -- 834-842 301/RConn1
  862/LConn3 -- 836-862 301/RConn3
  888/RConn1 -- 888-890 300/LConn1
  842/LConn3 -- 834-842 301/RConn3
  838 Y PQ/RConn1 -- Ground14/LConn1
  820Y Z/RConn1 -- Ground4/LConn1
  856 Y PQ/RConn1 -- Ground10/LConn1
  854 Y PQ/RConn1 -- Ground9/LConn1
  836/LConn1 -- 836 D PQ/LConn1 -- 860-836 301/RConn1
  "848 "/RConn3 -- 848 D PQ/LConn3 -- 848 Y Z/LConn3
  842-844 301/RConn3 -- 844/LConn3
  858 Y PQ/RConn1 -- Ground12/LConn1
  864 Y PQ/RConn1 -- Ground11/LConn1
  820 Y PQ/RConn1 -- Ground5/LConn1
  842-844 301/RConn2 -- 844/LConn2
  810 Y I/RConn1 -- Ground3/LConn1
  862 Y PQ/RConn1 -- Ground13/LConn1
  "848 "/RConn2 -- 848 D PQ/LConn2 -- 848 Y Z/LConn2
  862/LConn1 -- 836-862 301/RConn1
  824 Y I/RConn1 -- Ground7/LConn1
  862/LConn2 -- 836-862 301/RConn2
  826 Y I/RConn1 -- Ground8/LConn1
  840 Y I/LConn3 -- 840/RConn3
  808 Y I/RConn1 -- Ground1/LConn1
  "848 "/RConn1 -- 848 D PQ/LConn1 -- 848 Y Z/LConn1
  818 Y Z/RConn1 -- Ground2/LConn1
  844/LConn1 -- 844 Y PQ/LConn1 -- 842-844 301/RConn1
  822 Y PQ/RConn1 -- Ground6/LConn1
  860/RConn1 -- 860 Y PQ/LConn1 -- 860 D PQ/LConn1 -- 860-836 301/LConn1
  836/LConn2 -- 836 D PQ/LConn2 -- 860-836 301/RConn2
  860-836 301/LConn3 -- 860 D PQ/LConn3 -- 860 Y PQ/LConn3 -- 860/RConn3
  860-836 301/LConn2 -- 860 D PQ/LConn2 -- 860 Y PQ/LConn2 -- 860/RConn2
  840 Y I/LConn2 -- 840/RConn2
  836/LConn3 -- 836 D PQ/LConn3 -- 860-836 301/RConn3
  840 Y I/LConn1 -- 840/RConn1
  834/RConn3 -- 834 D Z/LConn3 -- 834-860 301/LConn3 -- 834-842 301/LConn3
  862/RConn2 -- 862 Y PQ/LConn1 -- 862-838 304/LConn1
  "816 "/LConn1 -- 850-816 301/RConn1
  840/LConn1 -- 840 D I/LConn1 -- 836-840 301/RConn1
  858-834 301/RConn3 -- 834 D PQ/LConn3 -- 834/LConn3
  834/LConn2 -- 834 D PQ/LConn2 -- 858-834 301/RConn2
  834/LConn1 -- 834 D PQ/LConn1 -- 858-834 301/RConn1
  840/LConn2 -- 840 D I/LConn2 -- 836-840 301/RConn2
  858 D Z/LConn3 -- 858/RConn3 -- 858 D PQ/LConn3 -- 858-834 301/LConn3
  840/LConn3 -- 840 D I/LConn3 -- 836-840 301/RConn3
  854-852 301/LConn3 -- 854/RConn3
  854-852 301/LConn1 -- 854/RConn1
  "816 "/LConn2 -- 850-816 301/RConn2
  "816 "/LConn3 -- 850-816 301/RConn3
  854 Y PQ/LConn1 -- 854-856 303/LConn1 -- 854-852 301/LConn2 -- 854/RConn2
  836-840 301/LConn2 -- 836 D I/LConn2 -- 836/RConn2 -- 836-862 301/LConn2
  836-840 301/LConn1 -- 836 D I/LConn1 -- 836-862 301/LConn1 -- 836/RConn1
  846-848 301/RConn3 -- "848 "/LConn3
  846-848 301/LConn3 -- 846/RConn3
  "848 "/LConn2 -- 848 Y PQ/LConn1 -- 846-848 301/RConn2
  836-840 301/LConn3 -- 836 D I/LConn3 -- 836/RConn3 -- 836-862 301/LConn3
  846-848 301/RConn1 -- "848 "/LConn1
  846/RConn2 -- 846 Y PQ1/LConn1 -- 846-848 301/LConn2
  834 D Z/LConn2 -- 834/RConn2 -- 834-860 301/LConn2 -- 834-842 301/LConn2
  834-860 301/RConn3 -- 860 D Z/LConn3 -- 860/LConn3
  854/LConn1 -- 830-854 301/RConn1
  834-860 301/LConn1 -- 834-842 301/LConn1 -- 834 D Z/LConn1 -- 834/RConn1
  842-844 301/LConn3 -- 842/RConn3
  854/LConn2 -- 830-854 301/RConn2
  846-848 301/LConn1 -- 846/RConn1
  858/LConn1 -- 832-858 301/RConn1
  844-846 301/LConn3 -- 844 Y PQ1/LConn3 -- 844 Y Z/LConn3 -- 844/RConn3 -- 844 Yg Z/LConn3
  842-844 301/LConn2 -- 842/RConn2
  844-846 301/LConn1 -- 844 Y PQ1/LConn1 -- 844 Y Z/LConn1 -- 844/RConn1 -- 844 Yg Z/LConn1
  858/LConn2 -- 832-858 301/RConn2
  854/LConn3 -- 830-854 301/RConn3
  842/RConn1 -- 842 Y PQ/LConn1 -- 842-844 301/LConn1
  834-860 301/RConn1 -- 860 D Z/LConn1 -- 860/LConn1
  830-854 301/LConn1 -- 830 D Z/LConn1 -- 830/RConn1
  830-854 301/LConn2 -- 830 D Z/LConn2 -- 830/RConn2
  846/LConn3 -- 846 Y PQ/LConn3 -- 844-846 301/RConn3
  846/LConn2 -- 846 Y PQ/LConn2 -- 844-846 301/RConn2
  858/LConn3 -- 832-858 301/RConn3
  844-846 301/LConn2 -- 844 Y PQ1/LConn2 -- 844 Y Z/LConn2 -- 844/RConn2 -- 844 Yg Z/LConn2
  830-854 301/LConn3 -- 830 D Z/LConn3 -- 830/RConn3
  834-860 301/RConn2 -- 860 D Z/LConn2 -- 860/LConn2
  846/LConn1 -- 846 Y PQ/LConn1 -- 844-846 301/RConn1
  818-820 302/LConn1 -- 818 Y Z/LConn1 -- 818/LConn1
  808/RConn3 -- 808-812 300/LConn3
  "816 "/RConn3 -- 816 D I/LConn3 -- 816-824 301/LConn3
  808/LConn3 -- 806-808 300/RConn3
  "816 "/RConn1 -- 816 D I/LConn1 -- 816-824 301/LConn1 -- 816-818 302/LConn1
  816-824 301/RConn3 -- 824 D I/LConn3 -- 824-828 301/LConn3 -- 826 Y I1/RConn1 -- "824 "/LConn3
  808/RConn1 -- 808-812 300/LConn1
  808/LConn2 -- 806-808 300/RConn2
  "824 "/RConn2 -- 824 Y I/LConn1 -- 824-826 303/LConn1
  828-830 301/LConn2 -- 828/RConn2
  830/LConn2 -- 828-830 301/RConn2
  808/RConn2 -- 808 Y I/LConn1 -- 808-810 303/LConn1 -- 808-812 300/LConn2
  820-822 302/LConn1 -- 820 Y PQ/LConn1 -- 820/LConn1
  828-830 301/LConn3 -- 828/RConn3
  816-824 301/LConn2 -- 816 D I/LConn2 -- "816 "/RConn2
  828/RConn1 -- 828 Y PQ1/LConn1 -- 828-830 301/LConn1
  824-828 301/RConn2 -- 828/LConn2
  830/LConn3 -- 828-830 301/RConn3
  824-828 301/RConn1 -- 828/LConn1
  824 D I/LConn2 -- 816-824 301/RConn2 -- 824-828 301/LConn2 -- "824 "/LConn2
  828-830 301/RConn1 -- 830 Y PQ/LConn1 -- 830/LConn1
  824-828 301/RConn3 -- 828 Y PQ/LConn1 -- 828/LConn3
  816-824 301/RConn1 -- 824 D I/LConn1 -- 824-828 301/LConn1 -- "824 "/LConn1
  806/LConn1 -- 802-806 300/RConn1
  802/RConn3 -- 802 Y PQ/LConn3 -- 802-806 300/LConn3
  802/LConn2 -- 800-802 300/RConn2
  806/RConn2 -- 806 Y PQ/LConn2 -- 806-808 300/LConn2
  806/RConn1 -- 806 Y PQ/LConn1 -- 806-808 300/LConn1
  806/LConn3 -- 802-806 300/RConn3
  802/RConn1 -- 802 Y PQ/LConn1 -- 802-806 300/LConn1
  808/LConn1 -- 806-808 300/RConn1
  802/LConn3 -- 800-802 300/RConn3
  802/RConn2 -- 802 Y PQ/LConn2 -- 802-806 300/LConn2
  806/RConn3 -- 806 Y PQ/LConn3 -- 806-808 300/LConn3
  806/LConn2 -- 802-806 300/RConn2
  802/LConn1 -- 800-802 300/RConn1
  Ground15/LConn1 -- 826 Y I1/LConn1
  Ground16/LConn1 -- 828 Y PQ/RConn1
  Ground17/LConn1 -- 828 Y PQ1/RConn1
  Ground18/LConn1 -- 830 Y PQ/RConn1
  Ground20/LConn1 -- 842 Y PQ/RConn1
  Ground19/LConn1 -- 844 Y PQ/RConn1
  Ground22/LConn1 -- 846 Y PQ1/RConn1
  Ground21/LConn1 -- 848 Y PQ/RConn1
  854-852 301/RConn1 -- "852 "/LConn1
  854-852 301/RConn2 -- "852 "/LConn2
  854-852 301/RConn3 -- "852 "/LConn3
  Three-Phase Transformer (Two Windings)1/RConn1 -- XF10/LConn1
  Three-Phase Transformer (Two Windings)1/RConn2 -- XF10/LConn2
  Three-Phase Transformer (Two Windings)1/RConn3 -- XF10/LConn3
